simulink model "IEEE30_case"  (R2024b)
settings: Solver=FixedStepAuto  StartTime=0  StopTime=5  FixedStep=1e-7  RelTol=1e-3
values from neighbouring files (symbols this model uses):
  GFL_DFIG_7_C_bus = 0.08    [IEEE30_case_parameters.m]
  GFL_DFIG_7_D_mutual = 2.500000e+3    (= 2500)    [IEEE30_case_parameters.m]
  GFL_DFIG_7_f0 = 60    [IEEE30_case_parameters.m]
  GFL_DFIG_7_gPLLi = 3200    [IEEE30_case_parameters.m]
  GFL_DFIG_7_gPLLp = 650    [IEEE30_case_parameters.m]
  GFL_DFIG_7_H_WT = 0.4    [IEEE30_case_parameters.m]
  GFL_DFIG_7_Hg = 0.8    [IEEE30_case_parameters.m]
  GFL_DFIG_7_Igq_ref = 0    [IEEE30_case_parameters.m]
  GFL_DFIG_7_Ird_ref = 704.45696    [IEEE30_case_parameters.m]
  GFL_DFIG_7_KI_V = -300000    [IEEE30_case_parameters.m]
  GFL_DFIG_7_KP_V = -1000    [IEEE30_case_parameters.m]
  GFL_DFIG_7_Ksh = 1.254300e+4    (= 12543)    [IEEE30_case_parameters.m]
  GFL_DFIG_7_Lg = 0.000483    [IEEE30_case_parameters.m]
  GFL_DFIG_7_Lm_pu = 4    [IEEE30_case_parameters.m]
  GFL_DFIG_7_N = 100    [IEEE30_case_parameters.m]
  GFL_DFIG_7_p = 2    [IEEE30_case_parameters.m]
  GFL_DFIG_7_Pitch = 0    [IEEE30_case_parameters.m]
  GFL_DFIG_7_R = 44    [IEEE30_case_parameters.m]
  GFL_DFIG_7_Rg = 2.000000e-5    (= 2e-05)    [IEEE30_case_parameters.m]
  GFL_DFIG_7_rho = 1.225    [IEEE30_case_parameters.m]
  GFL_DFIG_7_rPLLi = 4500    [IEEE30_case_parameters.m]
  GFL_DFIG_7_rPLLp = 620    [IEEE30_case_parameters.m]
  GFL_DFIG_7_Rs_pu = 0.011    [IEEE30_case_parameters.m]
  GFL_DFIG_7_Sbase = 2.000000e+6    (= 2000000)    [IEEE30_case_parameters.m]
  GFL_DFIG_7_ugq_ref = 0    [IEEE30_case_parameters.m]
  GFL_DFIG_7_usd_ref = 0    [IEEE30_case_parameters.m]
  GFL_DFIG_7_Vbase = 690    [IEEE30_case_parameters.m]
  GFL_DFIG_7_Vdc_ref = 1200    [IEEE30_case_parameters.m]
  GFL_DFIG_7_wind = 12    [IEEE30_case_parameters.m]
  GFL_DFIG_7_wm_ref = 518.184209    [IEEE30_case_parameters.m]
  SG_D_13_D = 0.01056    [IEEE30_case_parameters.m]
  SG_D_13_EnableSaturation = 0    [IEEE30_case_parameters.m]
  SG_D_13_f0 = 60    [IEEE30_case_parameters.m]
  SG_D_13_H = 7.5    [IEEE30_case_parameters.m]
  SG_D_13_K_A = 20    [IEEE30_case_parameters.m]
  SG_D_13_K_E = 1.000000e+1    (= 10)    [IEEE30_case_parameters.m]
  SG_D_13_K_F = 2.363    [IEEE30_case_parameters.m]
  SG_D_13_K_s = 0.5    [IEEE30_case_parameters.m]
  SG_D_13_R_a = 0.001088    [IEEE30_case_parameters.m]
  SG_D_13_S_A = 1    [IEEE30_case_parameters.m]
  SG_D_13_S_B = 0.103    [IEEE30_case_parameters.m]
  SG_D_13_S_N = 10.659857    [IEEE30_case_parameters.m]
  SG_D_13_SpeedPara = 200    [IEEE30_case_parameters.m]
  SG_D_13_T_0 = 0.370163    [IEEE30_case_parameters.m]
  SG_D_13_T_1 = 0.3    [IEEE30_case_parameters.m]
  SG_D_13_T_2 = 0.05    [IEEE30_case_parameters.m]
  SG_D_13_T_3 = 0.02    [IEEE30_case_parameters.m]
  SG_D_13_T_4 = 0.005    [IEEE30_case_parameters.m]
  SG_D_13_T_A = 0.02    [IEEE30_case_parameters.m]
  SG_D_13_T_dd = 8.000000e+0    (= 8)    [IEEE30_case_parameters.m]
  SG_D_13_T_ddd = 0.04    [IEEE30_case_parameters.m]
  SG_D_13_T_E = 0.314    [IEEE30_case_parameters.m]
  SG_D_13_T_F = 0.35    [IEEE30_case_parameters.m]
  SG_D_13_T_qd = 0.8    [IEEE30_case_parameters.m]
  SG_D_13_T_qdd = 0.02    [IEEE30_case_parameters.m]
  SG_D_13_T_speed = 0.1    [IEEE30_case_parameters.m]
  SG_D_13_T_w = 0.5    [IEEE30_case_parameters.m]
  SG_D_13_V_ref = 1.696619    [IEEE30_case_parameters.m]
  SG_D_13_w_ref = 376.991118    [IEEE30_case_parameters.m]
  SG_D_13_x_d = 1.9    [IEEE30_case_parameters.m]
  SG_D_13_x_dd = 0.302    [IEEE30_case_parameters.m]
  SG_D_13_x_ddd = 0.204    [IEEE30_case_parameters.m]
  SG_D_13_x_l = 0.05    [IEEE30_case_parameters.m]
  SG_D_13_x_q = 1.3    [IEEE30_case_parameters.m]
  SG_D_13_x_qd = 0.5    [IEEE30_case_parameters.m]
  SG_D_13_x_qdd = 0.3    [IEEE30_case_parameters.m]
  SG_D_1_D = 0.01056    [IEEE30_case_parameters.m]
  SG_D_1_EnableSaturation = 0    [IEEE30_case_parameters.m]
  SG_D_1_f0 = 60    [IEEE30_case_parameters.m]
  SG_D_1_H = 7.5    [IEEE30_case_parameters.m]
  SG_D_1_K_A = 20    [IEEE30_case_parameters.m]
  SG_D_1_K_E = 1.000000e+1    (= 10)    [IEEE30_case_parameters.m]
  SG_D_1_K_F = 2.363    [IEEE30_case_parameters.m]
  SG_D_1_K_s = 0.5    [IEEE30_case_parameters.m]
  SG_D_1_R_a = 0.001088    [IEEE30_case_parameters.m]
  SG_D_1_S_A = 1    [IEEE30_case_parameters.m]
  SG_D_1_S_B = 0.103    [IEEE30_case_parameters.m]
  SG_D_1_S_N = 10.659857    [IEEE30_case_parameters.m]
  SG_D_1_SpeedPara = 200    [IEEE30_case_parameters.m]
  SG_D_1_T_0 = 0.259812    [IEEE30_case_parameters.m]
  SG_D_1_T_1 = 0.3    [IEEE30_case_parameters.m]
  SG_D_1_T_2 = 0.05    [IEEE30_case_parameters.m]
  SG_D_1_T_3 = 0.02    [IEEE30_case_parameters.m]
  SG_D_1_T_4 = 0.005    [IEEE30_case_parameters.m]
  SG_D_1_T_A = 0.02    [IEEE30_case_parameters.m]
  SG_D_1_T_dd = 8.000000e+0    (= 8)    [IEEE30_case_parameters.m]
  SG_D_1_T_ddd = 0.04    [IEEE30_case_parameters.m]
  SG_D_1_T_E = 0.314    [IEEE30_case_parameters.m]
  SG_D_1_T_F = 0.35    [IEEE30_case_parameters.m]
  SG_D_1_T_qd = 0.8    [IEEE30_case_parameters.m]
  SG_D_1_T_qdd = 0.02    [IEEE30_case_parameters.m]
  SG_D_1_T_speed = 0.1    [IEEE30_case_parameters.m]
  SG_D_1_T_w = 0.5    [IEEE30_case_parameters.m]
  SG_D_1_V_ref = 1.544107    [IEEE30_case_parameters.m]
  SG_D_1_w_ref = 376.991118    [IEEE30_case_parameters.m]
  SG_D_1_x_d = 1.9    [IEEE30_case_parameters.m]
  SG_D_1_x_dd = 0.302    [IEEE30_case_parameters.m]
  SG_D_1_x_ddd = 0.204    [IEEE30_case_parameters.m]
  SG_D_1_x_l = 0.05    [IEEE30_case_parameters.m]
  SG_D_1_x_q = 1.3    [IEEE30_case_parameters.m]
  SG_D_1_x_qd = 0.5    [IEEE30_case_parameters.m]
  SG_D_1_x_qdd = 0.3    [IEEE30_case_parameters.m]
  SG_D_22_D = 0.01056    [IEEE30_case_parameters.m]
  SG_D_22_EnableSaturation = 0    [IEEE30_case_parameters.m]
  SG_D_22_f0 = 60    [IEEE30_case_parameters.m]
  SG_D_22_H = 7.5    [IEEE30_case_parameters.m]
  SG_D_22_K_A = 20    [IEEE30_case_parameters.m]
  SG_D_22_K_E = 1.000000e+1    (= 10)    [IEEE30_case_parameters.m]
  SG_D_22_K_F = 2.363    [IEEE30_case_parameters.m]
  SG_D_22_K_s = 0.5    [IEEE30_case_parameters.m]
  SG_D_22_R_a = 0.001088    [IEEE30_case_parameters.m]
  SG_D_22_S_A = 1    [IEEE30_case_parameters.m]
  SG_D_22_S_B = 0.103    [IEEE30_case_parameters.m]
  SG_D_22_S_N = 10.659857    [IEEE30_case_parameters.m]
  SG_D_22_SpeedPara = 200    [IEEE30_case_parameters.m]
  SG_D_22_T_0 = 0.216121    [IEEE30_case_parameters.m]
  SG_D_22_T_1 = 0.3    [IEEE30_case_parameters.m]
  SG_D_22_T_2 = 0.05    [IEEE30_case_parameters.m]
  SG_D_22_T_3 = 0.02    [IEEE30_case_parameters.m]
  SG_D_22_T_4 = 0.005    [IEEE30_case_parameters.m]
  ... (+126 more)
(part 2 of 27)

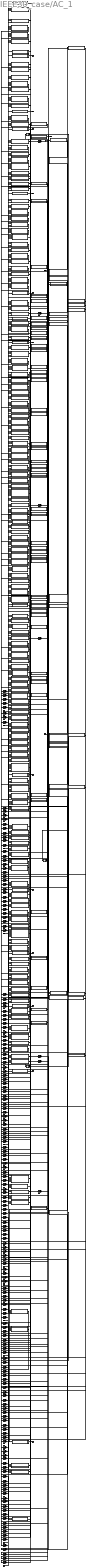
== system IEEE30_case/AC_1 ==
  id_SG_D_1 : Inport
  iq_SG_D_1 : Inport  Port=2
  id_SG_D_2 : Inport  Port=3
  iq_SG_D_2 : Inport  Port=4
  id_GFL_DFIG_7 : Inport  Port=5
  iq_GFL_DFIG_7 : Inport  Port=6
  id_SG_D_13 : Inport  Port=7
  iq_SG_D_13 : Inport  Port=8
  id_SG_D_22 : Inport  Port=9
  iq_SG_D_22 : Inport  Port=10
  id_SG_D_23 : Inport  Port=11
  iq_SG_D_23 : Inport  Port=12
  id_SG_D_27 : Inport  Port=13
  iq_SG_D_27 : Inport  Port=14
  d_id_line_10_17_block : Subsystem
  d_id_line_10_20_block : Subsystem
  d_id_line_10_21_block : Subsystem
  d_id_line_10_22_block : Subsystem
  d_id_line_12_13_block : Subsystem
  d_id_line_12_14_block : Subsystem
  d_id_line_12_15_block : Subsystem
  d_id_line_12_16_block : Subsystem
  d_id_line_14_15_block : Subsystem
  d_id_line_15_18_block : Subsystem
  d_id_line_15_23_block : Subsystem
  d_id_line_16_17_block : Subsystem
  d_id_line_18_19_block : Subsystem
  d_id_line_19_20_block : Subsystem
  d_id_line_1_2_block : Subsystem
  d_id_line_1_3_block : Subsystem
  d_id_line_21_22_block : Subsystem
  d_id_line_22_24_block : Subsystem
  d_id_line_23_24_block : Subsystem
  d_id_line_24_25_block : Subsystem
  d_id_line_25_26_block : Subsystem
  d_id_line_25_27_block : Subsystem
  d_id_line_27_29_block : Subsystem
  d_id_line_27_30_block : Subsystem
  d_id_line_28_27_block : Subsystem
  d_id_line_29_30_block : Subsystem
  d_id_line_2_4_block : Subsystem
  d_id_line_2_5_block : Subsystem
  d_id_line_2_6_block : Subsystem
  d_id_line_3_4_block : Subsystem
  d_id_line_4_12_block : Subsystem
  d_id_line_4_6_block : Subsystem
  d_id_line_5_7_block : Subsystem
  d_id_line_6_10_block : Subsystem
  d_id_line_6_28_block : Subsystem
  d_id_line_6_7_block : Subsystem
  d_id_line_6_8_block : Subsystem
  d_id_line_6_9_block : Subsystem
  d_id_line_8_28_block : Subsystem
  d_id_line_9_10_block : Subsystem
  d_id_line_9_11_block : Subsystem
  d_id_load_10_block : Subsystem
  d_id_load_12_block : Subsystem
  d_id_load_14_block : Subsystem
  d_id_load_15_block : Subsystem
  d_id_load_16_block : Subsystem
  d_id_load_17_block : Subsystem
  d_id_load_18_block : Subsystem
  d_id_load_19_block : Subsystem
  d_id_load_20_block : Subsystem
  d_id_load_21_block : Subsystem
  d_id_load_23_block : Subsystem
  d_id_load_24_block : Subsystem
  d_id_load_26_block : Subsystem
  d_id_load_29_block : Subsystem
  d_id_load_2_block : Subsystem
  d_id_load_30_block : Subsystem
  d_id_load_3_block : Subsystem
  d_id_load_4_block : Subsystem
  d_id_load_7_block : Subsystem
  d_id_load_8_block : Subsystem
  d_iq_line_10_17_block : Subsystem
  d_iq_line_10_20_block : Subsystem
  d_iq_line_10_21_block : Subsystem
  d_iq_line_10_22_block : Subsystem
  d_iq_line_12_13_block : Subsystem
  d_iq_line_12_14_block : Subsystem
  d_iq_line_12_15_block : Subsystem
  d_iq_line_12_16_block : Subsystem
  d_iq_line_14_15_block : Subsystem
  d_iq_line_15_18_block : Subsystem
  d_iq_line_15_23_block : Subsystem
  d_iq_line_16_17_block : Subsystem
  d_iq_line_18_19_block : Subsystem
  d_iq_line_19_20_block : Subsystem
  d_iq_line_1_2_block : Subsystem
  d_iq_line_1_3_block : Subsystem
  d_iq_line_21_22_block : Subsystem
  d_iq_line_22_24_block : Subsystem
  d_iq_line_23_24_block : Subsystem
  d_iq_line_24_25_block : Subsystem
  d_iq_line_25_26_block : Subsystem
  d_iq_line_25_27_block : Subsystem
  d_iq_line_27_29_block : Subsystem
  d_iq_line_27_30_block : Subsystem
  d_iq_line_28_27_block : Subsystem
  d_iq_line_29_30_block : Subsystem
  d_iq_line_2_4_block : Subsystem
  d_iq_line_2_5_block : Subsystem
  d_iq_line_2_6_block : Subsystem
  d_iq_line_3_4_block : Subsystem
  d_iq_line_4_12_block : Subsystem
  d_iq_line_4_6_block : Subsystem
  d_iq_line_5_7_block : Subsystem
  d_iq_line_6_10_block : Subsystem
  d_iq_line_6_28_block : Subsystem
  d_iq_line_6_7_block : Subsystem
  d_iq_line_6_8_block : Subsystem
  d_iq_line_6_9_block : Subsystem
  d_iq_line_8_28_block : Subsystem
  d_iq_line_9_10_block : Subsystem
  d_iq_line_9_11_block : Subsystem
  d_iq_load_10_block : Subsystem
  d_iq_load_12_block : Subsystem
  d_iq_load_14_block : Subsystem
  d_iq_load_15_block : Subsystem
  d_iq_load_16_block : Subsystem
  d_iq_load_17_block : Subsystem
  d_iq_load_18_block : Subsystem
  d_iq_load_19_block : Subsystem
  d_iq_load_20_block : Subsystem
  d_iq_load_21_block : Subsystem
  d_iq_load_23_block : Subsystem
  d_iq_load_24_block : Subsystem
  d_iq_load_26_block : Subsystem
  d_iq_load_29_block : Subsystem
  d_iq_load_2_block : Subsystem
  d_iq_load_30_block : Subsystem
  d_iq_load_3_block : Subsystem
  d_iq_load_4_block : Subsystem
  d_iq_load_7_block : Subsystem
  d_iq_load_8_block : Subsystem
  d_vd_bus_10_block : Subsystem
  d_vd_bus_11_block : Subsystem
  d_vd_bus_12_block : Subsystem
  d_vd_bus_13_block : Subsystem
  d_vd_bus_14_block : Subsystem
  d_vd_bus_15_block : Subsystem
  d_vd_bus_16_block : Subsystem
  d_vd_bus_17_block : Subsystem
  d_vd_bus_18_block : Subsystem
  d_vd_bus_19_block : Subsystem
  d_vd_bus_1_block : Subsystem
  d_vd_bus_20_block : Subsystem
  d_vd_bus_21_block : Subsystem
  d_vd_bus_22_block : Subsystem
  d_vd_bus_23_block : Subsystem
  d_vd_bus_24_block : Subsystem
  d_vd_bus_25_block : Subsystem
  d_vd_bus_26_block : Subsystem
  d_vd_bus_27_block : Subsystem
  d_vd_bus_28_block : Subsystem
  d_vd_bus_29_block : Subsystem
  d_vd_bus_2_block : Subsystem
  d_vd_bus_30_block : Subsystem
  d_vd_bus_3_block : Subsystem
  d_vd_bus_4_block : Subsystem
  d_vd_bus_5_block : Subsystem
  d_vd_bus_6_block : Subsystem
  d_vd_bus_7_block : Subsystem
  d_vd_bus_8_block : Subsystem
  d_vd_bus_9_block : Subsystem
  d_vq_bus_10_block : Subsystem
  d_vq_bus_11_block : Subsystem
  d_vq_bus_12_block : Subsystem
  d_vq_bus_13_block : Subsystem
  d_vq_bus_14_block : Subsystem
  d_vq_bus_15_block : Subsystem
  d_vq_bus_16_block : Subsystem
  d_vq_bus_17_block : Subsystem
  d_vq_bus_18_block : Subsystem
  d_vq_bus_19_block : Subsystem
  d_vq_bus_1_block : Subsystem
  d_vq_bus_20_block : Subsystem
  d_vq_bus_21_block : Subsystem
  d_vq_bus_22_block : Subsystem
  d_vq_bus_23_block : Subsystem
  d_vq_bus_24_block : Subsystem
  d_vq_bus_25_block : Subsystem
  d_vq_bus_26_block : Subsystem
  d_vq_bus_27_block : Subsystem
  d_vq_bus_28_block : Subsystem
  d_vq_bus_29_block : Subsystem
  d_vq_bus_2_block : Subsystem
  d_vq_bus_30_block : Subsystem
  d_vq_bus_3_block : Subsystem
  d_vq_bus_4_block : Subsystem
  d_vq_bus_5_block : Subsystem
  d_vq_bus_6_block : Subsystem
  d_vq_bus_7_block : Subsystem
  d_vq_bus_8_block : Subsystem
  d_vq_bus_9_block : Subsystem
  id_bus_10_block : Subsystem
  id_bus_11_block : Subsystem
  id_bus_12_block : Subsystem
  id_bus_13_block : Subsystem
  id_bus_14_block : Subsystem
  id_bus_15_block : Subsystem
  id_bus_16_block : Subsystem
  id_bus_17_block : Subsystem
  id_bus_18_block : Subsystem
  id_bus_19_block : Subsystem
  id_bus_1_block : Subsystem
  id_bus_20_block : Subsystem
  id_bus_21_block : Subsystem
  id_bus_22_block : Subsystem
  id_bus_23_block : Subsystem
  id_bus_24_block : Subsystem
  id_bus_25_block : Subsystem
  id_bus_26_block : Subsystem
  id_bus_27_block : Subsystem
  id_bus_28_block : Subsystem
  id_bus_29_block : Subsystem
  id_bus_2_block : Subsystem
  id_bus_30_block : Subsystem
  id_bus_3_block : Subsystem
  id_bus_4_block : Subsystem
  id_bus_5_block : Subsystem
  id_bus_6_block : Subsystem
  id_bus_7_block : Subsystem
  id_bus_8_block : Subsystem
  id_bus_9_block : Subsystem
  id_line_10_17 : Integrator  InitialCondition=0.0294
  id_line_10_20 : Integrator  InitialCondition=0.0572
  id_line_10_21 : Integrator  InitialCondition=-0.0157
  id_line_10_22 : Integrator  InitialCondition=-0.033
  id_line_12_13 : Integrator  InitialCondition=-0.3728
  id_line_12_14 : Integrator  InitialCondition=0.0544
  id_line_12_15 : Integrator  InitialCondition=0.0964
  id_line_12_16 : Integrator  InitialCondition=0.094
  id_line_14_15 : Integrator  InitialCondition=-0.0084
  id_line_15_18 : Integrator  InitialCondition=0.0931
  id_line_15_23 : Integrator  InitialCondition=-0.0876
  id_line_16_17 : Integrator  InitialCondition=0.0591
  id_line_18_19 : Integrator  InitialCondition=0.0607
  id_line_19_20 : Integrator  InitialCondition=-0.0351
  id_line_1_2 : Integrator  InitialCondition=0.1089
  id_line_1_3 : Integrator  InitialCondition=0.1508
  id_line_21_22 : Integrator  InitialCondition=-0.1847
  id_line_22_24 : Integrator  InitialCondition=-0.0256
  id_line_23_24 : Integrator  InitialCondition=0.0706
  id_line_24_25 : Integrator  InitialCondition=-0.0398
  id_line_25_26 : Integrator  InitialCondition=0.0351
  id_line_25_27 : Integrator  InitialCondition=-0.0749
  id_line_27_29 : Integrator  InitialCondition=0.0615
  id_line_27_30 : Integrator  InitialCondition=0.071
  id_line_28_27 : Integrator  InitialCondition=-0.0602
  id_line_29_30 : Integrator  InitialCondition=0.0373
  id_line_2_4 : Integrator  InitialCondition=0.1602
  id_line_2_5 : Integrator  InitialCondition=0.1375
  id_line_2_6 : Integrator  InitialCondition=0.2021
  id_line_3_4 : Integrator  InitialCondition=0.1265
  id_line_4_12 : Integrator  InitialCondition=-0.0164
  id_line_4_6 : Integrator  InitialCondition=0.2258
  id_line_5_7 : Integrator  InitialCondition=0.137
  id_line_6_10 : Integrator  InitialCondition=0.0347
  id_line_6_28 : Integrator  InitialCondition=-0.007
  id_line_6_7 : Integrator  InitialCondition=0.0937
  id_line_6_8 : Integrator  InitialCondition=0.2449
  id_line_6_9 : Integrator  InitialCondition=0.0608
  id_line_8_28 : Integrator  InitialCondition=-0.0526
  id_line_9_10 : Integrator  InitialCondition=0.0608
  id_line_9_11 : Integrator  InitialCondition=0.0
  id_load_10 : Integrator  InitialCondition=0.05762064982199419
  id_load_12 : Integrator  InitialCondition=0.11156942833231305
  id_load_14 : Integrator  InitialCondition=0.06276933195309545
  id_load_15 : Integrator  InitialCondition=0.08255703677859036
  id_load_16 : Integrator  InitialCondition=0.03492161173939187
  id_load_17 : Integrator  InitialCondition=0.08845667800489554
  id_load_18 : Integrator  InitialCondition=0.03241810454985263
  id_load_19 : Integrator  InitialCondition=0.09575018801243466
  id_load_2 : Integrator  InitialCondition=0.21607333892385353
  id_load_20 : Integrator  InitialCondition=0.02216052273204651
  id_load_21 : Integrator  InitialCondition=0.16897904373299158
  id_load_23 : Integrator  InitialCondition=0.031543951844660426
  id_load_24 : Integrator  InitialCondition=0.08480178555101445
  id_load_26 : Integrator  InitialCondition=0.03509280097479722
  id_load_29 : Integrator  InitialCondition=0.024141745519164363
  id_load_3 : Integrator  InitialCondition=0.024078796739266696
  id_load_30 : Integrator  InitialCondition=0.10832152401242767
  id_load_4 : Integrator  InitialCondition=0.07699434378766279
  id_load_7 : Integrator  InitialCondition=0.33349238327258734
  id_load_8 : Integrator  InitialCondition=0.29709225448369286
  iq_bus_10_block : Subsystem
  iq_bus_11_block : Subsystem
  iq_bus_12_block : Subsystem
  iq_bus_13_block : Subsystem
  iq_bus_14_block : Subsystem
  iq_bus_15_block : Subsystem
  iq_bus_16_block : Subsystem
  iq_bus_17_block : Subsystem
  iq_bus_18_block : Subsystem
  iq_bus_19_block : Subsystem
  iq_bus_1_block : Subsystem
  iq_bus_20_block : Subsystem
  iq_bus_21_block : Subsystem
  iq_bus_22_block : Subsystem
  iq_bus_23_block : Subsystem
  iq_bus_24_block : Subsystem
  iq_bus_25_block : Subsystem
  iq_bus_26_block : Subsystem
  iq_bus_27_block : Subsystem
  iq_bus_28_block : Subsystem
  iq_bus_29_block : Subsystem
  iq_bus_2_block : Subsystem
  iq_bus_30_block : Subsystem
  iq_bus_3_block : Subsystem
  iq_bus_4_block : Subsystem
  iq_bus_5_block : Subsystem
  iq_bus_6_block : Subsystem
  iq_bus_7_block : Subsystem
  iq_bus_8_block : Subsystem
  iq_bus_9_block : Subsystem
  iq_line_10_17 : Integrator  InitialCondition=-0.0833
  iq_line_10_20 : Integrator  InitialCondition=-0.0504
  iq_line_10_21 : Integrator  InitialCondition=0.1196
  iq_line_10_22 : Integrator  InitialCondition=0.0883
  iq_line_12_13 : Integrator  InitialCondition=0.104
  iq_line_12_14 : Integrator  InitialCondition=-0.0104
  iq_line_12_15 : Integrator  InitialCondition=0.0082
  iq_line_12_16 : Integrator  InitialCondition=-0.0015
  iq_line_14_15 : Integrator  InitialCondition=0.0085
  iq_line_15_18 : Integrator  InitialCondition=-0.0115
  iq_line_15_23 : Integrator  InitialCondition=0.0571
  iq_line_16_17 : Integrator  InitialCondition=0.0186
  iq_line_18_19 : Integrator  InitialCondition=-0.0002
  iq_line_19_20 : Integrator  InitialCondition=0.0417
  iq_line_1_2 : Integrator  InitialCondition=0.0359
  iq_line_1_3 : Integrator  InitialCondition=-0.0509
  iq_line_21_22 : Integrator  InitialCondition=0.2429
  iq_line_22_24 : Integrator  InitialCondition=-0.0766
  iq_line_23_24 : Integrator  InitialCondition=-0.0108
  iq_line_24_25 : Integrator  InitialCondition=-0.0161
  iq_line_25_26 : Integrator  InitialCondition=-0.025
  iq_line_25_27 : Integrator  InitialCondition=0.0089
  iq_line_27_29 : Integrator  InitialCondition=-0.0177
  iq_line_27_30 : Integrator  InitialCondition=-0.0178
  iq_line_28_27 : Integrator  InitialCondition=0.0649
  iq_line_29_30 : Integrator  InitialCondition=-0.0076
  iq_line_2_4 : Integrator  InitialCondition=-0.0632
  iq_line_2_5 : Integrator  InitialCondition=-0.0561
  iq_line_2_6 : Integrator  InitialCondition=-0.0857
  iq_line_3_4 : Integrator  InitialCondition=-0.0479
  iq_line_4_12 : Integrator  InitialCondition=0.0212
  iq_line_4_6 : Integrator  InitialCondition=-0.1233
  iq_line_5_7 : Integrator  InitialCondition=-0.0727
  iq_line_6_10 : Integrator  InitialCondition=0.0183
  iq_line_6_28 : Integrator  InitialCondition=0.0232
  iq_line_6_7 : Integrator  InitialCondition=-0.0411
  iq_line_6_8 : Integrator  InitialCondition=-0.2609
  iq_line_6_9 : Integrator  InitialCondition=0.0321
  iq_line_8_28 : Integrator  InitialCondition=0.0563
  iq_line_9_10 : Integrator  InitialCondition=0.0321
  iq_line_9_11 : Integrator  InitialCondition=0.0
  iq_load_10 : Integrator  InitialCondition=-0.023750155710290172
  iq_load_12 : Integrator  InitialCondition=-0.07912681099168954
  iq_load_14 : Integrator  InitialCondition=-0.018925276841010825
  iq_load_15 : Integrator  InitialCondition=-0.028857933169465035
  iq_load_16 : Integrator  InitialCondition=-0.02004887361778872
  iq_load_17 : Integrator  InitialCondition=-0.06472122976436909
  iq_load_18 : Integrator  InitialCondition=-0.011280947855116687
  iq_load_19 : Integrator  InitialCondition=-0.041932223185470595
  iq_load_2 : Integrator  InitialCondition=-0.12857026174935463
  iq_load_20 : Integrator  InitialCondition=-0.008738712343444175
  iq_load_21 : Integrator  InitialCondition=-0.12325613888050702
  iq_load_23 : Integrator  InitialCondition=-0.016881324060089138
  iq_load_24 : Integrator  InitialCondition=-0.07174395043107668
  iq_load_26 : Integrator  InitialCondition=-0.024985253536549745
  iq_load_29 : Integrator  InitialCondition=-0.010091059482716875
  iq_load_3 : Integrator  InitialCondition=-0.01284992759642887
  iq_load_30 : Integrator  InitialCondition=-0.025413778164099808
  iq_load_4 : Integrator  InitialCondition=-0.018745546356930477
  iq_load_7 : Integrator  InitialCondition=-0.1282452809846534
  iq_load_8 : Integrator  InitialCondition=-0.3267952741267314
  vd_bus_1 : Integrator  InitialCondition=1.0
  vd_bus_10 : Integrator  InitialCondition=0.9826970239916736
  vd_bus_11 : Integrator  InitialCondition=0.9791651158395024
  vd_bus_12 : Integrator  InitialCondition=0.9851138013134092
  vd_bus_13 : Integrator  InitialCondition=0.9996681288543109
  vd_bus_13_out_block : Subsystem
  vd_bus_14 : Integrator  InitialCondition=0.9758845077744954
  vd_bus_15 : Integrator  InitialCondition=0.9794312058156106
  vd_bus_16 : Integrator  InitialCondition=0.9763547800086462
  vd_bus_17 : Integrator  InitialCondition=0.9751536962265143
  vd_bus_18 : Integrator  InitialCondition=0.9666562258898125
  vd_bus_19 : Integrator  InitialCondition=0.9629845116632844
  vd_bus_1_out_block : Subsystem
  vd_bus_2 : Integrator  InitialCondition=0.9999737066760137
  vd_bus_20 : Integrator  InitialCondition=0.96695524349606
  vd_bus_21 : Integrator  InitialCondition=0.9915427046125346
  vd_bus_22 : Integrator  InitialCondition=0.998247346015286
  vd_bus_22_out_block : Subsystem
  vd_bus_23 : Integrator  InitialCondition=0.9996153468676248
  vd_bus_23_out_block : Subsystem
  vd_bus_24 : Integrator  InitialCondition=0.9875238668019122
  vd_bus_25 : Integrator  InitialCondition=0.9897841246173575
  vd_bus_26 : Integrator  InitialCondition=0.9715165251247116
  vd_bus_27 : Integrator  InitialCondition=0.9998954705679283
  vd_bus_27_out_block : Subsystem
  vd_bus_28 : Integrator  InitialCondition=0.9739527539680385
  vd_bus_29 : Integrator  InitialCondition=0.9789208214366218
  vd_bus_2_out_block : Subsystem
  vd_bus_3 : Integrator  InitialCondition=0.9827914051679246
  vd_bus_30 : Integrator  InitialCondition=0.9665194654171512
  vd_bus_4 : Integrator  InitialCondition=0.9796122119954275
  vd_bus_5 : Integrator  InitialCondition=0.9818864593128205
  vd_bus_6 : Integrator  InitialCondition=0.9724223804183465
  vd_bus_7 : Integrator  InitialCondition=0.9663195284431091
  vd_bus_7_out_block : Subsystem
  vd_bus_8 : Integrator  InitialCondition=0.9595368480969235
  vd_bus_9 : Integrator  InitialCondition=0.9791651158395024
  vq_bus_1 : Integrator  InitialCondition=0.0
  vq_bus_10 : Integrator  InitialCondition=-0.05795157371804589
  vq_bus_11 : Integrator  InitialCondition=-0.051263313202214764
  vq_bus_12 : Integrator  InitialCondition=-0.026431197200791515
  vq_bus_13 : Integrator  InitialCondition=0.02576105884704402
  vq_bus_13_out_block : Subsystem
  vq_bus_14 : Integrator  InitialCondition=-0.039332654939370465
  vq_bus_15 : Integrator  InitialCondition=-0.03954066677889769
  vq_bus_16 : Integrator  InitialCondition=-0.04509567319714669
  vq_bus_17 : Integrator  InitialCondition=-0.057803961717475
  vq_bus_18 : Integrator  InitialCondition=-0.05875724397019161
  vq_bus_19 : Integrator  InitialCondition=-0.0666325737803011
  vq_bus_1_out_block : Subsystem
  vq_bus_2 : Integrator  InitialCondition=-0.007251617518437124
  vq_bus_20 : Integrator  InitialCondition=-0.06542912996363182
  vq_bus_21 : Integrator  InitialCondition=-0.06044373953148359
  vq_bus_22 : Integrator  InitialCondition=-0.059179693928221304
  vq_bus_22_out_block : Subsystem
  vq_bus_23 : Integrator  InitialCondition=-0.02773370344397317
  vq_bus_23_out_block : Subsystem
  vq_bus_24 : Integrator  InitialCondition=-0.045386583835857836
  vq_bus_25 : Integrator  InitialCondition=-0.029203013743050087
  vq_bus_26 : Integrator  InitialCondition=-0.036291964728132654
  vq_bus_27 : Integrator  InitialCondition=-0.014458490161195933
  vq_bus_27_out_block : Subsystem
  vq_bus_28 : Integrator  InitialCondition=-0.03853789459848076
  vq_bus_29 : Integrator  InitialCondition=-0.036382963166013
  vq_bus_2_out_block : Subsystem
  vq_bus_3 : Integrator  InitialCondition=-0.026114195223675894
  vq_bus_30 : Integrator  InitialCondition=-0.05135554854968241
  vq_bus_4 : Integrator  InitialCondition=-0.030695321441965278
  vq_bus_5 : Integrator  InitialCondition=-0.03195188283298677
  vq_bus_6 : Integrator  InitialCondition=-0.038494815818198067
  vq_bus_7 : Integrator  InitialCondition=-0.04475640282897933
  vq_bus_7_out_block : Subsystem
  vq_bus_8 : Integrator  InitialCondition=-0.04568314085508728
  vq_bus_9 : Integrator  InitialCondition=-0.051263313202214764
  vd_bus_1_out : Outport
  vq_bus_1_out : Outport  Port=2
  vd_bus_2_out : Outport  Port=3
  vq_bus_2_out : Outport  Port=4
  vd_bus_7_out : Outport  Port=5
  vq_bus_7_out : Outport  Port=6
  vd_bus_13_out : Outport  Port=7
  vq_bus_13_out : Outport  Port=8
  vd_bus_22_out : Outport  Port=9
  vq_bus_22_out : Outport  Port=10
  vd_bus_23_out : Outport  Port=11
  vq_bus_23_out : Outport  Port=12
  vd_bus_27_out : Outport  Port=13
  vq_bus_27_out : Outport  Port=14
  wires:
  id_line_2_6/1 -> id_bus_6_block/1(State_id_line_2_6_f1c81), id_bus_2_block/6(State_id_line_2_6_b437f), d_id_line_2_6_block/1(State_id_line_2_6_7d8f0), d_iq_line_2_6_block/1(State_id_line_2_6_7b42f)
  id_SG_D_27/1 -> id_bus_27_block/1(Input_id_SG_D_27_bfa21)
  iq_line_27_29/1 -> d_id_line_27_29_block/2(State_iq_line_27_29_70df7), d_iq_line_27_29_block/2(State_iq_line_27_29_e2b12), iq_bus_27_block/3(State_iq_line_27_29_e7090), iq_bus_29_block/2(State_iq_line_27_29_eb40a)
  iq_line_2_5/1 -> d_id_line_2_5_block/2(State_iq_line_2_5_6b567), iq_bus_2_block/5(State_iq_line_2_5_9d19f), d_iq_line_2_5_block/2(State_iq_line_2_5_e8b89), iq_bus_5_block/1(State_iq_line_2_5_98d2b)
  iq_SG_D_27/1 -> iq_bus_27_block/1(Input_iq_SG_D_27_5f248)
  id_bus_4_block/1(Blockout_id_bus_4_62c4e) -> d_vd_bus_4_block/1(Alge_id_bus_4_472b5)
  id_line_12_13/1 -> d_iq_line_12_13_block/1(State_id_line_12_13_e0b57), id_bus_12_block/3(State_id_line_12_13_02bcf), id_bus_13_block/2(State_id_line_12_13_e1ea8)
  iq_line_28_27/1 -> iq_bus_27_block/5(State_iq_line_28_27_c8698), iq_bus_28_block/3(State_iq_line_28_27_5cab2), d_id_line_28_27_block/1(State_iq_line_28_27_dccca)
  id_load_19/1 -> d_iq_load_19_block/1(State_id_load_19_a4f80), d_id_load_19_block/1(State_id_load_19_86caa), id_bus_19_block/1(State_id_load_19_6dd0b)
  iq_load_19/1 -> d_id_load_19_block/2(State_iq_load_19_76cc3), iq_bus_19_block/1(State_iq_load_19_c9423), d_iq_load_19_block/2(State_iq_load_19_a3943)
  d_id_line_22_24_block/1(Blockout_d_id_line_22_24_ad4cf) -> id_line_22_24/1
  iq_line_1_2/1 -> iq_bus_1_block/2(State_iq_line_1_2_426df), iq_bus_2_block/3(State_iq_line_1_2_22297), d_id_line_1_2_block/2(State_iq_line_1_2_034b5), d_iq_line_1_2_block/2(State_iq_line_1_2_62f2c)
  iq_GFL_DFIG_7/1 -> iq_bus_7_block/1(Input_iq_GFL_DFIG_7_603eb)
  id_bus_10_block/1(Blockout_id_bus_10_f7cfc) -> d_vd_bus_10_block/1(Alge_id_bus_10_55824)
  vq_bus_25/1 -> d_iq_line_25_26_block/3(State_vq_bus_25_a69b5), d_iq_line_24_25_block/4(State_vq_bus_25_584b4), d_vd_bus_25_block/2(State_vq_bus_25_926f5), d_iq_line_25_27_block/3(State_vq_bus_25_cd5c7)
  d_vq_bus_26_block/1(Blockout_d_vq_bus_26_2e68a) -> vq_bus_26/1
  iq_SG_D_23/1 -> iq_bus_23_block/1(Input_iq_SG_D_23_15e34)
  iq_SG_D_22/1 -> iq_bus_22_block/1(Input_iq_SG_D_22_7afaf)
  iq_bus_13_block/1(Blockout_iq_bus_13_72f64) -> d_vq_bus_13_block/1(Alge_iq_bus_13_8e98b)
  id_bus_9_block/1(Blockout_id_bus_9_0b36c) -> d_vd_bus_9_block/1(Alge_id_bus_9_9bb77)
  d_id_load_4_block/1(Blockout_d_id_load_4_41d2b) -> id_load_4/1
  id_bus_12_block/1(Blockout_id_bus_12_a7f7d) -> d_vd_bus_12_block/1(Alge_id_bus_12_e0ed8)
  d_vd_bus_21_block/1(Blockout_d_vd_bus_21_3eacf) -> vd_bus_21/1
  d_iq_line_6_28_block/1(Blockout_d_iq_line_6_28_5907d) -> iq_line_6_28/1
  id_line_27_30/1 -> d_id_line_27_30_block/1(State_id_line_27_30_d82b5), d_iq_line_27_30_block/1(State_id_line_27_30_d18cd), id_bus_30_block/2(State_id_line_27_30_55115), id_bus_27_block/4(State_id_line_27_30_1b75b)
  id_bus_25_block/1(Blockout_id_bus_25_a9e73) -> d_vd_bus_25_block/1(Alge_id_bus_25_c584c)
  vd_bus_2_out_block/1(Blockout_vd_bus_2_out_6e542) -> vd_bus_2_out/1
  d_id_load_16_block/1(Blockout_d_id_load_16_4c50d) -> id_load_16/1
  iq_load_4/1 -> d_id_load_4_block/2(State_iq_load_4_59598), iq_bus_4_block/1(State_iq_load_4_0a7a4), d_iq_load_4_block/2(State_iq_load_4_cbd44)
  d_vq_bus_13_block/1(Blockout_d_vq_bus_13_29628) -> vq_bus_13/1
  id_load_18/1 -> id_bus_18_block/1(State_id_load_18_b6089), d_id_load_18_block/1(State_id_load_18_c255f), d_iq_load_18_block/1(State_id_load_18_cc435)
  iq_line_25_27/1 -> iq_bus_27_block/2(State_iq_line_25_27_786f4), iq_bus_25_block/3(State_iq_line_25_27_6cee1), d_id_line_25_27_block/2(State_iq_line_25_27_73a3b), d_iq_line_25_27_block/2(State_iq_line_25_27_e5d71)
  id_bus_18_block/1(Blockout_id_bus_18_f6aba) -> d_vd_bus_18_block/1(Alge_id_bus_18_7cead)
  d_iq_load_7_block/1(Blockout_d_iq_load_7_f7ad2) -> iq_load_7/1
  d_vd_bus_18_block/1(Blockout_d_vd_bus_18_c0af9) -> vd_bus_18/1
  d_iq_line_4_12_block/1(Blockout_d_iq_line_4_12_9b276) -> iq_line_4_12/1
  id_line_1_2/1 -> d_iq_line_1_2_block/1(State_id_line_1_2_bca8d), id_bus_1_block/2(State_id_line_1_2_dfc68), d_id_line_1_2_block/1(State_id_line_1_2_ffdd4), id_bus_2_block/3(State_id_line_1_2_35b9f)
  id_line_1_3/1 -> d_id_line_1_3_block/1(State_id_line_1_3_6eb6f), id_bus_1_block/3(State_id_line_1_3_6e2c0), id_bus_3_block/2(State_id_line_1_3_85a3c), d_iq_line_1_3_block/1(State_id_line_1_3_ae183)
  id_GFL_DFIG_7/1 -> id_bus_7_block/1(Input_id_GFL_DFIG_7_848f8)
  id_SG_D_13/1 -> id_bus_13_block/1(Input_id_SG_D_13_a3cac)
  d_id_line_6_8_block/1(Blockout_d_id_line_6_8_230ec) -> id_line_6_8/1
  iq_bus_19_block/1(Blockout_iq_bus_19_07988) -> d_vq_bus_19_block/1(Alge_iq_bus_19_ec54b)
  iq_bus_21_block/1(Blockout_iq_bus_21_51471) -> d_vq_bus_21_block/1(Alge_iq_bus_21_81fa7)
  d_iq_load_8_block/1(Blockout_d_iq_load_8_09960) -> iq_load_8/1
  id_bus_6_block/1(Blockout_id_bus_6_41f21) -> d_vd_bus_6_block/1(Alge_id_bus_6_cc19e)
  iq_load_26/1 -> d_iq_load_26_block/2(State_iq_load_26_73904), iq_bus_26_block/1(State_iq_load_26_ac2a5), d_id_load_26_block/2(State_iq_load_26_8de5f)
  id_SG_D_22/1 -> id_bus_22_block/1(Input_id_SG_D_22_c72e9)
  d_vq_bus_14_block/1(Blockout_d_vq_bus_14_01909) -> vq_bus_14/1
  id_bus_3_block/1(Blockout_id_bus_3_36e80) -> d_vd_bus_3_block/1(Alge_id_bus_3_320e9)
  id_SG_D_23/1 -> id_bus_23_block/1(Input_id_SG_D_23_b9b6b)
  d_iq_line_19_20_block/1(Blockout_d_iq_line_19_20_abe71) -> iq_line_19_20/1
  d_id_line_9_10_block/1(Blockout_d_id_line_9_10_c8100) -> id_line_9_10/1
  vq_bus_28/1 -> d_vd_bus_28_block/2(State_vq_bus_28_2c3ac), d_iq_line_28_27_block/3(State_vq_bus_28_55731), d_iq_line_6_28_block/3(State_vq_bus_28_c063c), d_iq_line_8_28_block/3(State_vq_bus_28_2fdab)
  vq_bus_29/1 -> d_vd_bus_29_block/2(State_vq_bus_29_f75e0), d_iq_line_29_30_block/3(State_vq_bus_29_3e7b3), d_iq_load_29_block/3(State_vq_bus_29_603a8), d_iq_line_27_29_block/4(State_vq_bus_29_394c9)
  vq_bus_16/1 -> d_vd_bus_16_block/2(State_vq_bus_16_133e3), d_iq_line_12_16_block/4(State_vq_bus_16_185e6), d_iq_load_16_block/3(State_vq_bus_16_c51f8), d_iq_line_16_17_block/3(State_vq_bus_16_312ae)
  iq_bus_8_block/1(Blockout_iq_bus_8_3c8c0) -> d_vq_bus_8_block/1(Alge_iq_bus_8_bb8a6)
  d_id_line_16_17_block/1(Blockout_d_id_line_16_17_1cf66) -> id_line_16_17/1
  iq_line_2_6/1 -> d_id_line_2_6_block/2(State_iq_line_2_6_13ccb), iq_bus_2_block/6(State_iq_line_2_6_42b8c), iq_bus_6_block/1(State_iq_line_2_6_0b501), d_iq_line_2_6_block/2(State_iq_line_2_6_17b05)
  iq_line_6_28/1 -> iq_bus_6_block/7(State_iq_line_6_28_c6c23), d_iq_line_6_28_block/2(State_iq_line_6_28_bd7e8), d_id_line_6_28_block/2(State_iq_line_6_28_4e6de), iq_bus_28_block/1(State_iq_line_6_28_9fc56)
  id_SG_D_1/1 -> id_bus_1_block/1(Input_id_SG_D_1_df3b6)
  id_load_29/1 -> d_id_load_29_block/1(State_id_load_29_75998), id_bus_29_block/1(State_id_load_29_01b75), d_iq_load_29_block/1(State_id_load_29_0ee5a)
  id_line_22_24/1 -> d_id_line_22_24_block/1(State_id_line_22_24_bf52a), id_bus_24_block/2(State_id_line_22_24_03003), d_iq_line_22_24_block/1(State_id_line_22_24_f3c92), id_bus_22_block/4(State_id_line_22_24_1a6a9)
  d_id_line_18_19_block/1(Blockout_d_id_line_18_19_39807) -> id_line_18_19/1
  iq_load_14/1 -> d_id_load_14_block/2(State_iq_load_14_d649f), d_iq_load_14_block/2(State_iq_load_14_32f4c), iq_bus_14_block/1(State_iq_load_14_72e79)
  iq_bus_28_block/1(Blockout_iq_bus_28_fc1de) -> d_vq_bus_28_block/1(Alge_iq_bus_28_e3380)
  vd_bus_1/1 -> d_vq_bus_1_block/2(State_vd_bus_1_0a414), vd_bus_1_out_block/1(State_vd_bus_1_2d719), d_id_line_1_2_block/3(State_vd_bus_1_c4c37), d_id_line_1_3_block/3(State_vd_bus_1_5ec44)
  d_iq_load_18_block/1(Blockout_d_iq_load_18_ea1d4) -> iq_load_18/1
  d_vq_bus_3_block/1(Blockout_d_vq_bus_3_10f19) -> vq_bus_3/1
  d_iq_line_22_24_block/1(Blockout_d_iq_line_22_24_c0f91) -> iq_line_22_24/1
  iq_SG_D_13/1 -> iq_bus_13_block/1(Input_iq_SG_D_13_41b6f)
  d_id_line_10_21_block/1(Blockout_d_id_line_10_21_8be6c) -> id_line_10_21/1
  vq_bus_2/1 -> d_vd_bus_2_block/2(State_vq_bus_2_2b9b5), d_iq_line_1_2_block/4(State_vq_bus_2_54dcd), d_iq_line_2_5_block/3(State_vq_bus_2_03b90), vq_bus_2_out_block/1(State_vq_bus_2_331ca), d_iq_line_2_4_block/3(State_vq_bus_2_08b2a), d_iq_line_2_6_block/3(State_vq_bus_2_0704f), d_iq_load_2_block/3(State_vq_bus_2_2efc8)
  vd_bus_29/1 -> d_vq_bus_29_block/2(State_vd_bus_29_8221e), d_id_line_29_30_block/3(State_vd_bus_29_072b3), d_id_line_27_29_block/4(State_vd_bus_29_a9de4), d_id_load_29_block/3(State_vd_bus_29_01a46)
  d_vd_bus_16_block/1(Blockout_d_vd_bus_16_30db1) -> vd_bus_16/1
  iq_bus_30_block/1(Blockout_iq_bus_30_f5578) -> d_vq_bus_30_block/1(Alge_iq_bus_30_b84d2)
  iq_line_8_28/1 -> d_id_line_8_28_block/2(State_iq_line_8_28_05745), d_iq_line_8_28_block/2(State_iq_line_8_28_65df2), iq_bus_8_block/3(State_iq_line_8_28_57c78), iq_bus_28_block/2(State_iq_line_8_28_5df2a)
  id_load_24/1 -> d_id_load_24_block/1(State_id_load_24_1ae10), d_iq_load_24_block/1(State_id_load_24_9d769), id_bus_24_block/1(State_id_load_24_1483c)
  id_load_14/1 -> d_id_load_14_block/1(State_id_load_14_cc3a3), d_iq_load_14_block/1(State_id_load_14_258e7), id_bus_14_block/1(State_id_load_14_8acb6)
  d_iq_load_30_block/1(Blockout_d_iq_load_30_29807) -> iq_load_30/1
  iq_line_22_24/1 -> d_id_line_22_24_block/2(State_iq_line_22_24_ef354), iq_bus_22_block/4(State_iq_line_22_24_573df), iq_bus_24_block/2(State_iq_line_22_24_76281), d_iq_line_22_24_block/2(State_iq_line_22_24_cd212)
  d_iq_load_26_block/1(Blockout_d_iq_load_26_2c5ef) -> iq_load_26/1
  vq_bus_27/1 -> d_vd_bus_27_block/2(State_vq_bus_27_1ff45), d_iq_line_25_27_block/4(State_vq_bus_27_3c154), d_iq_line_27_29_block/3(State_vq_bus_27_cc3b8), d_iq_line_27_30_block/3(State_vq_bus_27_cb66b), vq_bus_27_out_block/1(State_vq_bus_27_50cd3), d_iq_line_28_27_block/2(State_vq_bus_27_b0dc4)
  id_bus_16_block/1(Blockout_id_bus_16_3e58c) -> d_vd_bus_16_block/1(Alge_id_bus_16_f0bf0)
  id_line_14_15/1 -> d_id_line_14_15_block/1(State_id_line_14_15_28cb1), d_iq_line_14_15_block/1(State_id_line_14_15_7494d), id_bus_15_block/3(State_id_line_14_15_22f97), id_bus_14_block/3(State_id_line_14_15_8760d)
  d_id_line_10_20_block/1(Blockout_d_id_line_10_20_f93f3) -> id_line_10_20/1
  iq_bus_29_block/1(Blockout_iq_bus_29_54fcd) -> d_vq_bus_29_block/1(Alge_iq_bus_29_a773e)
  vq_bus_20/1 -> d_iq_line_19_20_block/4(State_vq_bus_20_72c0e), d_vd_bus_20_block/2(State_vq_bus_20_f55e8), d_iq_load_20_block/3(State_vq_bus_20_5757f), d_iq_line_10_20_block/4(State_vq_bus_20_32cb1)
  d_iq_line_9_11_block/1(Blockout_d_iq_line_9_11_ec45f) -> iq_line_9_11/1
  d_iq_line_25_26_block/1(Blockout_d_iq_line_25_26_d7e2d) -> iq_line_25_26/1
  d_vq_bus_10_block/1(Blockout_d_vq_bus_10_d65a2) -> vq_bus_10/1
  id_bus_20_block/1(Blockout_id_bus_20_0c62a) -> d_vd_bus_20_block/1(Alge_id_bus_20_5519e)
  iq_load_30/1 -> iq_bus_30_block/1(State_iq_load_30_e4c4c), d_id_load_30_block/2(State_iq_load_30_241a5), d_iq_load_30_block/2(State_iq_load_30_a149a)
  iq_SG_D_1/1 -> iq_bus_1_block/1(Input_iq_SG_D_1_636be)
  iq_SG_D_2/1 -> iq_bus_2_block/1(Input_iq_SG_D_2_3deae)
  id_line_10_22/1 -> id_bus_10_block/7(State_id_line_10_22_301e1), id_bus_22_block/2(State_id_line_10_22_83f91), d_id_line_10_22_block/1(State_id_line_10_22_89fbc), d_iq_line_10_22_block/1(State_id_line_10_22_084f6)
  id_SG_D_2/1 -> id_bus_2_block/1(Input_id_SG_D_2_271b9)
  id_load_8/1 -> d_id_load_8_block/1(State_id_load_8_d111e), d_iq_load_8_block/1(State_id_load_8_a69c1), id_bus_8_block/1(State_id_load_8_2d300)
  iq_line_10_22/1 -> d_id_line_10_22_block/2(State_iq_line_10_22_73dd3), iq_bus_10_block/7(State_iq_line_10_22_b2379), d_iq_line_10_22_block/2(State_iq_line_10_22_3080a), iq_bus_22_block/2(State_iq_line_10_22_172f8)
  id_bus_19_block/1(Blockout_id_bus_19_c959d) -> d_vd_bus_19_block/1(Alge_id_bus_19_2b5fc)
  id_load_15/1 -> d_id_load_15_block/1(State_id_load_15_eb719), id_bus_15_block/1(State_id_load_15_060ab), d_iq_load_15_block/1(State_id_load_15_529a5)
  iq_line_23_24/1 -> d_id_line_23_24_block/2(State_iq_line_23_24_865cb), iq_bus_23_block/4(State_iq_line_23_24_17ece), iq_bus_24_block/3(State_iq_line_23_24_946d1), d_iq_line_23_24_block/2(State_iq_line_23_24_146a4)
  id_load_2/1 -> d_id_load_2_block/1(State_id_load_2_b9eb3), d_iq_load_2_block/1(State_id_load_2_4fe58), id_bus_2_block/2(State_id_load_2_17a4a)
  iq_line_19_20/1 -> d_id_line_19_20_block/2(State_iq_line_19_20_aecba), iq_bus_19_block/3(State_iq_line_19_20_3626a), d_iq_line_19_20_block/2(State_iq_line_19_20_2451d), iq_bus_20_block/3(State_iq_line_19_20_435ec)
  id_bus_30_block/1(Blockout_id_bus_30_50341) -> d_vd_bus_30_block/1(Alge_id_bus_30_9d0e0)
  id_bus_7_block/1(Blockout_id_bus_7_1a1e5) -> d_vd_bus_7_block/1(Alge_id_bus_7_b77de)
  id_bus_11_block/1(Blockout_id_bus_11_04e0f) -> d_vd_bus_11_block/1(Alge_id_bus_11_02d21)
  vd_bus_30/1 -> d_id_load_30_block/3(State_vd_bus_30_c111a), d_id_line_29_30_block/4(State_vd_bus_30_f5954), d_id_line_27_30_block/4(State_vd_bus_30_fc433), d_vq_bus_30_block/2(State_vd_bus_30_536bd)
  iq_bus_14_block/1(Blockout_iq_bus_14_40877) -> d_vq_bus_14_block/1(Alge_iq_bus_14_fa60c)
  iq_line_18_19/1 -> d_iq_line_18_19_block/2(State_iq_line_18_19_da0b4), iq_bus_18_block/3(State_iq_line_18_19_1de76), iq_bus_19_block/2(State_iq_line_18_19_b0a61), d_id_line_18_19_block/2(State_iq_line_18_19_bad0a)
  id_line_5_7/1 -> d_id_line_5_7_block/1(State_id_line_5_7_f4de4), d_iq_line_5_7_block/1(State_id_line_5_7_c3a9a), id_bus_5_block/2(State_id_line_5_7_98a48), id_bus_7_block/3(State_id_line_5_7_86c29)
  id_bus_22_block/1(Blockout_id_bus_22_34fe4) -> d_vd_bus_22_block/1(Alge_id_bus_22_6e14d)
  iq_load_7/1 -> d_iq_load_7_block/2(State_iq_load_7_42ee7), iq_bus_7_block/2(State_iq_load_7_52d26), d_id_load_7_block/2(State_iq_load_7_25d21)
  id_bus_15_block/1(Blockout_id_bus_15_03e1f) -> d_vd_bus_15_block/1(Alge_id_bus_15_5fc28)
  id_bus_29_block/1(Blockout_id_bus_29_dcea9) -> d_vd_bus_29_block/1(Alge_id_bus_29_eb4d1)
  d_vd_bus_28_block/1(Blockout_d_vd_bus_28_2c5eb) -> vd_bus_28/1
  iq_line_1_3/1 -> iq_bus_1_block/3(State_iq_line_1_3_a1a02), iq_bus_3_block/2(State_iq_line_1_3_704f9), d_iq_line_1_3_block/2(State_iq_line_1_3_f4510), d_id_line_1_3_block/2(State_iq_line_1_3_e0dcf)
  d_iq_load_16_block/1(Blockout_d_iq_load_16_0762f) -> iq_load_16/1
  iq_load_15/1 -> d_iq_load_15_block/2(State_iq_load_15_0f08a), iq_bus_15_block/1(State_iq_load_15_d1891), d_id_load_15_block/2(State_iq_load_15_a3946)
  iq_line_6_7/1 -> d_iq_line_6_7_block/2(State_iq_line_6_7_562f8), iq_bus_7_block/4(State_iq_line_6_7_6dde0), d_id_line_6_7_block/2(State_iq_line_6_7_8098b), iq_bus_6_block/3(State_iq_line_6_7_5270c)
  id_bus_28_block/1(Blockout_id_bus_28_5bbbe) -> d_vd_bus_28_block/1(Alge_id_bus_28_5e372)
  d_iq_load_24_block/1(Blockout_d_iq_load_24_ad216) -> iq_load_24/1
  d_vq_bus_22_block/1(Blockout_d_vq_bus_22_04fe2) -> vq_bus_22/1
  d_iq_line_12_15_block/1(Blockout_d_iq_line_12_15_872fa) -> iq_line_12_15/1
  id_line_15_23/1 -> d_iq_line_15_23_block/1(State_id_line_15_23_e0160), d_id_line_15_23_block/1(State_id_line_15_23_5b9f7), id_bus_15_block/5(State_id_line_15_23_df0bc), id_bus_23_block/3(State_id_line_15_23_e01a5)
  iq_bus_27_block/1(Blockout_iq_bus_27_6c5f3) -> d_vq_bus_27_block/1(Alge_iq_bus_27_548e5)
  iq_load_29/1 -> d_iq_load_29_block/2(State_iq_load_29_c7734), iq_bus_29_block/1(State_iq_load_29_82b4e), d_id_load_29_block/2(State_iq_load_29_726f9)
  id_bus_27_block/1(Blockout_id_bus_27_09b01) -> d_vd_bus_27_block/1(Alge_id_bus_27_de3da)
  vd_bus_7/1 -> d_vq_bus_7_block/2(State_vd_bus_7_0bd1f), d_id_load_7_block/3(State_vd_bus_7_efc9a), vd_bus_7_out_block/1(State_vd_bus_7_01f81), d_id_line_5_7_block/4(State_vd_bus_7_ca274), d_id_line_6_7_block/4(State_vd_bus_7_fcdb6)
  vd_bus_26/1 -> d_id_load_26_block/3(State_vd_bus_26_1ef7d), d_id_line_25_26_block/4(State_vd_bus_26_fc271), d_vq_bus_26_block/2(State_vd_bus_26_21468)
  iq_line_12_16/1 -> d_iq_line_12_16_block/2(State_iq_line_12_16_057ef), iq_bus_16_block/2(State_iq_line_12_16_8d22f), iq_bus_12_block/6(State_iq_line_12_16_bc787), d_id_line_12_16_block/2(State_iq_line_12_16_288fb)
  vd_bus_13_out_block/1(Blockout_vd_bus_13_out_de49d) -> vd_bus_13_out/1
  iq_bus_17_block/1(Blockout_iq_bus_17_f1a33) -> d_vq_bus_17_block/1(Alge_iq_bus_17_e57db)
  iq_bus_26_block/1(Blockout_iq_bus_26_d1a08) -> d_vq_bus_26_block/1(Alge_iq_bus_26_172b0)
  d_iq_line_6_8_block/1(Blockout_d_iq_line_6_8_b8ba9) -> iq_line_6_8/1
  vd_bus_6/1 -> d_vq_bus_6_block/2(State_vd_bus_6_1a151), d_id_line_4_6_block/4(State_vd_bus_6_4e65f), d_id_line_6_10_block/3(State_vd_bus_6_f8a31), d_id_line_6_7_block/3(State_vd_bus_6_7185e), d_id_line_2_6_block/4(State_vd_bus_6_4e456), d_id_line_6_8_block/3(State_vd_bus_6_a2a00), d_id_line_6_28_block/4(State_vd_bus_6_24f43), d_id_line_6_9_block/2(State_vd_bus_6_dd441)
  vd_bus_4/1 -> d_vq_bus_4_block/2(State_vd_bus_4_783ad), d_id_line_2_4_block/4(State_vd_bus_4_468ae), d_id_line_4_6_block/3(State_vd_bus_4_4594e), d_id_line_4_12_block/3(State_vd_bus_4_83c34), d_id_load_4_block/3(State_vd_bus_4_a96c2), d_id_line_3_4_block/4(State_vd_bus_4_76476)
  iq_bus_20_block/1(Blockout_iq_bus_20_faa95) -> d_vq_bus_20_block/1(Alge_iq_bus_20_dac44)
  d_vd_bus_30_block/1(Blockout_d_vd_bus_30_d4924) -> vd_bus_30/1
  vq_bus_4/1 -> d_vd_bus_4_block/2(State_vq_bus_4_40a27), d_iq_line_4_6_block/3(State_vq_bus_4_bd5e4), d_iq_load_4_block/3(State_vq_bus_4_cd35f), d_iq_line_2_4_block/4(State_vq_bus_4_bf96b), d_iq_line_4_12_block/3(State_vq_bus_4_bbada), d_iq_line_3_4_block/4(State_vq_bus_4_f5988)
  id_bus_1_block/1(Blockout_id_bus_1_c8a02) -> d_vd_bus_1_block/1(Alge_id_bus_1_1678c)
  id_bus_21_block/1(Blockout_id_bus_21_f6b53) -> d_vd_bus_21_block/1(Alge_id_bus_21_08784)
  d_vq_bus_28_block/1(Blockout_d_vq_bus_28_fc78f) -> vq_bus_28/1
  vq_bus_14/1 -> d_iq_load_14_block/3(State_vq_bus_14_0c5a3), d_iq_line_14_15_block/3(State_vq_bus_14_61922), d_vd_bus_14_block/2(State_vq_bus_14_a6726), d_iq_line_12_14_block/4(State_vq_bus_14_44cc5)
  id_bus_26_block/1(Blockout_id_bus_26_f258d) -> d_vd_bus_26_block/1(Alge_id_bus_26_ff4d0)
  iq_bus_25_block/1(Blockout_iq_bus_25_a2b76) -> d_vq_bus_25_block/1(Alge_iq_bus_25_b52f0)
  id_bus_13_block/1(Blockout_id_bus_13_e8139) -> d_vd_bus_13_block/1(Alge_id_bus_13_da285)
  iq_bus_24_block/1(Blockout_iq_bus_24_a8f54) -> d_vq_bus_24_block/1(Alge_iq_bus_24_0b825)
  iq_bus_4_block/1(Blockout_iq_bus_4_c8ef1) -> d_vq_bus_4_block/1(Alge_iq_bus_4_edea5)
  id_bus_24_block/1(Blockout_id_bus_24_85e6b) -> d_vd_bus_24_block/1(Alge_id_bus_24_d1ab9)
  d_iq_line_12_14_block/1(Blockout_d_iq_line_12_14_a9efb) -> iq_line_12_14/1
  vq_bus_23_out_block/1(Blockout_vq_bus_23_out_e2230) -> vq_bus_23_out/1
  iq_bus_23_block/1(Blockout_iq_bus_23_896ad) -> d_vq_bus_23_block/1(Alge_iq_bus_23_4fd9f)
  d_id_line_28_27_block/1(Blockout_d_id_line_28_27_ed70c) -> id_line_28_27/1
  id_bus_17_block/1(Blockout_id_bus_17_5f54e) -> d_vd_bus_17_block/1(Alge_id_bus_17_92d80)
  iq_line_9_10/1 -> d_id_line_9_10_block/1(State_iq_line_9_10_60482), iq_bus_10_block/3(State_iq_line_9_10_547ec), iq_bus_9_block/2(State_iq_line_9_10_59358)
  id_bus_23_block/1(Blockout_id_bus_23_84113) -> d_vd_bus_23_block/1(Alge_id_bus_23_3d01a)
  iq_line_15_23/1 -> d_id_line_15_23_block/2(State_iq_line_15_23_b33ff), iq_bus_15_block/5(State_iq_line_15_23_dd72a), iq_bus_23_block/3(State_iq_line_15_23_fc0a9), d_iq_line_15_23_block/2(State_iq_line_15_23_ade94)
  iq_bus_22_block/1(Blockout_iq_bus_22_6516e) -> d_vq_bus_22_block/1(Alge_iq_bus_22_4e114)
  d_id_line_23_24_block/1(Blockout_d_id_line_23_24_092ff) -> id_line_23_24/1
  vd_bus_17/1 -> d_vq_bus_17_block/2(State_vd_bus_17_b3717), d_id_line_16_17_block/4(State_vd_bus_17_81d16), d_id_line_10_17_block/4(State_vd_bus_17_0c9ca), d_id_load_17_block/3(State_vd_bus_17_34bc4)
  iq_line_24_25/1 -> d_id_line_24_25_block/2(State_iq_line_24_25_5d4c8), d_iq_line_24_25_block/2(State_iq_line_24_25_774ec), iq_bus_24_block/4(State_iq_line_24_25_99c0f), iq_bus_25_block/1(State_iq_line_24_25_0047e)
  iq_bus_18_block/1(Blockout_iq_bus_18_b4916) -> d_vq_bus_18_block/1(Alge_iq_bus_18_aa760)
  id_load_3/1 -> d_iq_load_3_block/1(State_id_load_3_67436), id_bus_3_block/1(State_id_load_3_6a44d), d_id_load_3_block/1(State_id_load_3_6ca3f)
  vd_bus_3/1 -> d_vq_bus_3_block/2(State_vd_bus_3_2475d), d_id_line_1_3_block/4(State_vd_bus_3_137a9), d_id_load_3_block/3(State_vd_bus_3_703c2), d_id_line_3_4_block/3(State_vd_bus_3_9cd0a)
  id_load_10/1 -> d_iq_load_10_block/1(State_id_load_10_13915), id_bus_10_block/1(State_id_load_10_705f8), d_id_load_10_block/1(State_id_load_10_b4421)
  id_line_6_10/1 -> d_iq_line_6_10_block/1(State_id_line_6_10_fd3de), id_bus_10_block/2(State_id_line_6_10_65dc9), id_bus_6_block/6(State_id_line_6_10_2c687)
  iq_bus_16_block/1(Blockout_iq_bus_16_0845b) -> d_vq_bus_16_block/1(Alge_iq_bus_16_974ba)
  d_vd_bus_8_block/1(Blockout_d_vd_bus_8_6724c) -> vd_bus_8/1
  iq_line_9_11/1 -> iq_bus_9_block/3(State_iq_line_9_11_56031), iq_bus_11_block/1(State_iq_line_9_11_5dafe), d_id_line_9_11_block/1(State_iq_line_9_11_d1a32)
  id_line_28_27/1 -> id_bus_27_block/5(State_id_line_28_27_22b40), id_bus_28_block/3(State_id_line_28_27_48f21), d_iq_line_28_27_block/1(State_id_line_28_27_3a5d8)
  iq_bus_12_block/1(Blockout_iq_bus_12_94dfd) -> d_vq_bus_12_block/1(Alge_iq_bus_12_c8c41)
  vq_bus_6/1 -> d_vd_bus_6_block/2(State_vq_bus_6_b1fab), d_iq_line_6_9_block/2(State_vq_bus_6_65d52), d_iq_line_6_10_block/3(State_vq_bus_6_fa482), d_iq_line_2_6_block/4(State_vq_bus_6_e98dc), d_iq_line_6_7_block/3(State_vq_bus_6_83d07), d_iq_line_4_6_block/4(State_vq_bus_6_b2fe0), d_iq_line_6_28_block/4(State_vq_bus_6_177ff), d_iq_line_6_8_block/3(State_vq_bus_6_241ca)
  d_vd_bus_6_block/1(Blockout_d_vd_bus_6_cb8a2) -> vd_bus_6/1
  iq_bus_15_block/1(Blockout_iq_bus_15_ccbd2) -> d_vq_bus_15_block/1(Alge_iq_bus_15_10184)
  d_iq_load_10_block/1(Blockout_d_iq_load_10_a5f74) -> iq_load_10/1
  id_line_10_21/1 -> id_bus_10_block/6(State_id_line_10_21_c8fce), id_bus_21_block/2(State_id_line_10_21_bcd00), d_iq_line_10_21_block/1(State_id_line_10_21_eaa10), d_id_line_10_21_block/1(State_id_line_10_21_d3f7b)
  d_id_line_9_11_block/1(Blockout_d_id_line_9_11_6700a) -> id_line_9_11/1
  vd_bus_9/1 -> d_id_line_9_11_block/3(State_vd_bus_9_653b8), d_id_line_9_10_block/3(State_vd_bus_9_a12d0), d_id_line_6_9_block/3(State_vd_bus_9_1e8eb), d_vq_bus_9_block/2(State_vd_bus_9_08774)
  id_bus_14_block/1(Blockout_id_bus_14_a7723) -> d_vd_bus_14_block/1(Alge_id_bus_14_c396c)
  d_vq_bus_6_block/1(Blockout_d_vq_bus_6_ac6cf) -> vq_bus_6/1
  d_iq_load_12_block/1(Blockout_d_iq_load_12_fd87b) -> iq_load_12/1
  d_vd_bus_9_block/1(Blockout_d_vd_bus_9_ffce9) -> vd_bus_9/1
  vd_bus_22_out_block/1(Blockout_vd_bus_22_out_b1115) -> vd_bus_22_out/1
  iq_bus_11_block/1(Blockout_iq_bus_11_40b0f) -> d_vq_bus_11_block/1(Alge_iq_bus_11_6efd4)
  id_line_6_9/1 -> id_bus_9_block/1(State_id_line_6_9_06348), id_bus_6_block/5(State_id_line_6_9_c95db), d_iq_line_6_9_block/1(State_id_line_6_9_7cf57)
  id_bus_2_block/1(Blockout_id_bus_2_bbec8) -> d_vd_bus_2_block/1(Alge_id_bus_2_79afc)
  id_load_26/1 -> d_id_load_26_block/1(State_id_load_26_7d329), id_bus_26_block/1(State_id_load_26_80bb7), d_iq_load_26_block/1(State_id_load_26_7e9e7)
  d_vq_bus_5_block/1(Blockout_d_vq_bus_5_f1f0c) -> vq_bus_5/1
  d_iq_line_2_6_block/1(Blockout_d_iq_line_2_6_890b3) -> iq_line_2_6/1
  iq_bus_10_block/1(Blockout_iq_bus_10_f080b) -> d_vq_bus_10_block/1(Alge_iq_bus_10_74e9d)
  d_vq_bus_12_block/1(Blockout_d_vq_bus_12_c4166) -> vq_bus_12/1
  iq_line_15_18/1 -> iq_bus_15_block/4(State_iq_line_15_18_a2738), d_id_line_15_18_block/2(State_iq_line_15_18_872e9), d_iq_line_15_18_block/2(State_iq_line_15_18_85966), iq_bus_18_block/2(State_iq_line_15_18_3f1e8)
  d_iq_line_23_24_block/1(Blockout_d_iq_line_23_24_07ba5) -> iq_line_23_24/1
  vd_bus_27_out_block/1(Blockout_vd_bus_27_out_73c03) -> vd_bus_27_out/1
  vd_bus_28/1 -> d_vq_bus_28_block/2(State_vd_bus_28_5e73c), d_id_line_28_27_block/3(State_vd_bus_28_9edc3), d_id_line_8_28_block/3(State_vd_bus_28_83ac0), d_id_line_6_28_block/3(State_vd_bus_28_34661)
  d_iq_line_25_27_block/1(Blockout_d_iq_line_25_27_06e15) -> iq_line_25_27/1
  id_bus_8_block/1(Blockout_id_bus_8_ac02c) -> d_vd_bus_8_block/1(Alge_id_bus_8_ddcea)
  vq_bus_10/1 -> d_iq_line_6_10_block/2(State_vq_bus_10_9c824), d_iq_line_10_20_block/3(State_vq_bus_10_01ccf), d_iq_load_10_block/3(State_vq_bus_10_c6f4b), d_iq_line_10_22_block/3(State_vq_bus_10_6b45e), d_vd_bus_10_block/2(State_vq_bus_10_0727d), d_iq_line_10_21_block/3(State_vq_bus_10_d2e20), d_iq_line_10_17_block/3(State_vq_bus_10_bd672), d_iq_line_9_10_block/2(State_vq_bus_10_72139)
  iq_bus_7_block/1(Blockout_iq_bus_7_06239) -> d_vq_bus_7_block/1(Alge_iq_bus_7_86528)
  iq_bus_6_block/1(Blockout_iq_bus_6_4f954) -> d_vq_bus_6_block/1(Alge_iq_bus_6_8f458)
  iq_bus_5_block/1(Blockout_iq_bus_5_aa6f8) -> d_vq_bus_5_block/1(Alge_iq_bus_5_20adf)
  id_bus_5_block/1(Blockout_id_bus_5_f0a59) -> d_vd_bus_5_block/1(Alge_id_bus_5_015f0)
  vq_bus_17/1 -> d_vd_bus_17_block/2(State_vq_bus_17_c3ce6), d_iq_line_10_17_block/4(State_vq_bus_17_4f180), d_iq_line_16_17_block/4(State_vq_bus_17_5c6e8), d_iq_load_17_block/3(State_vq_bus_17_aeaf0)
  d_id_line_10_17_block/1(Blockout_d_id_line_10_17_512b4) -> id_line_10_17/1
  d_id_line_10_22_block/1(Blockout_d_id_line_10_22_d0b41) -> id_line_10_22/1
  iq_load_24/1 -> d_id_load_24_block/2(State_iq_load_24_33ce7), d_iq_load_24_block/2(State_iq_load_24_562ce), iq_bus_24_block/1(State_iq_load_24_fdcb6)
  iq_bus_3_block/1(Blockout_iq_bus_3_0811d) -> d_vq_bus_3_block/1(Alge_iq_bus_3_cb5cd)
  iq_bus_2_block/1(Blockout_iq_bus_2_bb89e) -> d_vq_bus_2_block/1(Alge_iq_bus_2_6cf64)
  id_line_6_8/1 -> id_bus_6_block/4(State_id_line_6_8_8d48d), d_id_line_6_8_block/1(State_id_line_6_8_be2c2), d_iq_line_6_8_block/1(State_id_line_6_8_d622b), id_bus_8_block/2(State_id_line_6_8_e60f9)
  iq_bus_1_block/1(Blockout_iq_bus_1_c22d8) -> d_vq_bus_1_block/1(Alge_iq_bus_1_d0ef3)
  vd_bus_11/1 -> d_vq_bus_11_block/2(State_vd_bus_11_8616a), d_id_line_9_11_block/2(State_vd_bus_11_30158)
  iq_line_3_4/1 -> d_iq_line_3_4_block/2(State_iq_line_3_4_a2132), iq_bus_4_block/3(State_iq_line_3_4_5b109), iq_bus_3_block/3(State_iq_line_3_4_e67cb), d_id_line_3_4_block/2(State_iq_line_3_4_97dfa)
  id_line_25_26/1 -> d_iq_line_25_26_block/1(State_id_line_25_26_499e6), id_bus_26_block/2(State_id_line_25_26_45789), id_bus_25_block/2(State_id_line_25_26_94c65), d_id_line_25_26_block/1(State_id_line_25_26_99f78)
  vq_bus_27_out_block/1(Blockout_vq_bus_27_out_7c7b9) -> vq_bus_27_out/1
  id_line_15_18/1 -> d_id_line_15_18_block/1(State_id_line_15_18_9ff35), d_iq_line_15_18_block/1(State_id_line_15_18_c7b72), id_bus_18_block/2(State_id_line_15_18_185de), id_bus_15_block/4(State_id_line_15_18_9837d)
  vd_bus_23_out_block/1(Blockout_vd_bus_23_out_e84a6) -> vd_bus_23_out/1
  vd_bus_23/1 -> d_vq_bus_23_block/2(State_vd_bus_23_43c98), d_id_load_23_block/3(State_vd_bus_23_3d25c), d_id_line_23_24_block/3(State_vd_bus_23_dd709), d_id_line_15_23_block/4(State_vd_bus_23_ce9b8), vd_bus_23_out_block/1(State_vd_bus_23_a2fc7)
  iq_line_12_13/1 -> d_id_line_12_13_block/1(State_iq_line_12_13_e9023), iq_bus_13_block/2(State_iq_line_12_13_2e588), iq_bus_12_block/3(State_iq_line_12_13_64934)
  vq_bus_22_out_block/1(Blockout_vq_bus_22_out_dafa4) -> vq_bus_22_out/1
  vq_bus_13_out_block/1(Blockout_vq_bus_13_out_2bf25) -> vq_bus_13_out/1
  vd_bus_12/1 -> d_id_load_12_block/3(State_vd_bus_12_e073f), d_id_line_12_16_block/3(State_vd_bus_12_31adb), d_vq_bus_12_block/2(State_vd_bus_12_a627c), d_id_line_12_15_block/3(State_vd_bus_12_a4ba8), d_id_line_12_13_block/2(State_vd_bus_12_4b72e), d_id_line_4_12_block/2(State_vd_bus_12_eb3f5), d_id_line_12_14_block/3(State_vd_bus_12_691f6)
  iq_line_10_20/1 -> iq_bus_10_block/5(State_iq_line_10_20_d3f34), iq_bus_20_block/2(State_iq_line_10_20_d570b), d_iq_line_10_20_block/2(State_iq_line_10_20_af332), d_id_line_10_20_block/2(State_iq_line_10_20_a2259)
  id_line_21_22/1 -> d_iq_line_21_22_block/1(State_id_line_21_22_6fd19), id_bus_22_block/3(State_id_line_21_22_cc6ca), id_bus_21_block/3(State_id_line_21_22_cc9c2), d_id_line_21_22_block/1(State_id_line_21_22_e74c3)
  vq_bus_7_out_block/1(Blockout_vq_bus_7_out_1686e) -> vq_bus_7_out/1
  d_vd_bus_12_block/1(Blockout_d_vd_bus_12_8eaf3) -> vd_bus_12/1
  d_id_load_2_block/1(Blockout_d_id_load_2_a0af3) -> id_load_2/1
  vq_bus_23/1 -> d_vd_bus_23_block/2(State_vq_bus_23_506e6), vq_bus_23_out_block/1(State_vq_bus_23_75786), d_iq_load_23_block/3(State_vq_bus_23_fbc77), d_iq_line_23_24_block/3(State_vq_bus_23_d5a58), d_iq_line_15_23_block/4(State_vq_bus_23_32b73)
  vq_bus_1/1 -> d_vd_bus_1_block/2(State_vq_bus_1_acb41), d_iq_line_1_3_block/3(State_vq_bus_1_564cd), vq_bus_1_out_block/1(State_vq_bus_1_5ae62), d_iq_line_1_2_block/3(State_vq_bus_1_1d692)
  vq_bus_18/1 -> d_vd_bus_18_block/2(State_vq_bus_18_b1f41), d_iq_load_18_block/3(State_vq_bus_18_1cdbe), d_iq_line_15_18_block/4(State_vq_bus_18_6e5b1), d_iq_line_18_19_block/3(State_vq_bus_18_f4e53)
  vd_bus_7_out_block/1(Blockout_vd_bus_7_out_4e91c) -> vd_bus_7_out/1
  vq_bus_2_out_block/1(Blockout_vq_bus_2_out_9085b) -> vq_bus_2_out/1
  iq_line_27_30/1 -> d_id_line_27_30_block/2(State_iq_line_27_30_37807), d_iq_line_27_30_block/2(State_iq_line_27_30_e9a72), iq_bus_27_block/4(State_iq_line_27_30_e8aeb), iq_bus_30_block/2(State_iq_line_27_30_c3531)
  vq_bus_1_out_block/1(Blockout_vq_bus_1_out_7cf09) -> vq_bus_1_out/1
  iq_line_12_14/1 -> d_id_line_12_14_block/2(State_iq_line_12_14_78bfe), iq_bus_12_block/4(State_iq_line_12_14_05407), iq_bus_14_block/2(State_iq_line_12_14_c9961), d_iq_line_12_14_block/2(State_iq_line_12_14_89ecd)
  d_id_line_12_15_block/1(Blockout_d_id_line_12_15_9a1c2) -> id_line_12_15/1
  d_id_line_12_13_block/1(Blockout_d_id_line_12_13_70d92) -> id_line_12_13/1
  d_vq_bus_1_block/1(Blockout_d_vq_bus_1_b6261) -> vq_bus_1/1
  id_line_18_19/1 -> d_iq_line_18_19_block/1(State_id_line_18_19_8f9c3), id_bus_19_block/2(State_id_line_18_19_4e3a3), d_id_line_18_19_block/1(State_id_line_18_19_ee31e), id_bus_18_block/3(State_id_line_18_19_1fd25)
  d_vq_bus_7_block/1(Blockout_d_vq_bus_7_71b97) -> vq_bus_7/1
  vd_bus_1_out_block/1(Blockout_vd_bus_1_out_a0239) -> vd_bus_1_out/1
  iq_line_14_15/1 -> d_iq_line_14_15_block/2(State_iq_line_14_15_6bca3), d_id_line_14_15_block/2(State_iq_line_14_15_9579a), iq_bus_14_block/3(State_iq_line_14_15_62994), iq_bus_15_block/3(State_iq_line_14_15_cd3f2)
  vd_bus_27/1 -> d_vq_bus_27_block/2(State_vd_bus_27_e355a), d_id_line_25_27_block/4(State_vd_bus_27_199bb), d_id_line_27_30_block/3(State_vd_bus_27_614b7), d_id_line_27_29_block/3(State_vd_bus_27_91239), d_id_line_28_27_block/2(State_vd_bus_27_3c49b), vd_bus_27_out_block/1(State_vd_bus_27_9c8fe)
  iq_line_12_15/1 -> d_id_line_12_15_block/2(State_iq_line_12_15_08071), d_iq_line_12_15_block/2(State_iq_line_12_15_4b1af), iq_bus_12_block/5(State_iq_line_12_15_032f0), iq_bus_15_block/2(State_iq_line_12_15_d11d7)
  d_id_line_6_10_block/1(Blockout_d_id_line_6_10_40498) -> id_line_6_10/1
  vd_bus_21/1 -> d_vq_bus_21_block/2(State_vd_bus_21_a8899), d_id_line_21_22_block/3(State_vd_bus_21_3bbf1), d_id_load_21_block/3(State_vd_bus_21_5dea6), d_id_line_10_21_block/4(State_vd_bus_21_53c66)
  iq_line_5_7/1 -> d_id_line_5_7_block/2(State_iq_line_5_7_abaf2), iq_bus_5_block/2(State_iq_line_5_7_0b183), iq_bus_7_block/3(State_iq_line_5_7_dcfea), d_iq_line_5_7_block/2(State_iq_line_5_7_98783)
  vd_bus_15/1 -> d_vq_bus_15_block/2(State_vd_bus_15_568cb), d_id_load_15_block/3(State_vd_bus_15_8a842), d_id_line_15_18_block/3(State_vd_bus_15_67b4c), d_id_line_15_23_block/3(State_vd_bus_15_742a0), d_id_line_14_15_block/4(State_vd_bus_15_c6d58), d_id_line_12_15_block/4(State_vd_bus_15_2851a)
  d_id_line_27_30_block/1(Blockout_d_id_line_27_30_26949) -> id_line_27_30/1
  vq_bus_24/1 -> d_vd_bus_24_block/2(State_vq_bus_24_3465a), d_iq_line_24_25_block/3(State_vq_bus_24_1bac9), d_iq_line_22_24_block/4(State_vq_bus_24_1befd), d_iq_line_23_24_block/4(State_vq_bus_24_00c5d), d_iq_load_24_block/3(State_vq_bus_24_612f6)
  d_id_line_27_29_block/1(Blockout_d_id_line_27_29_5ee71) -> id_line_27_29/1
  iq_line_6_9/1 -> d_id_line_6_9_block/1(State_iq_line_6_9_a3af3), iq_bus_6_block/5(State_iq_line_6_9_51dc2), iq_bus_9_block/1(State_iq_line_6_9_55e22)
  vd_bus_18/1 -> d_vq_bus_18_block/2(State_vd_bus_18_3c890), d_id_load_18_block/3(State_vd_bus_18_bf8f3), d_id_line_18_19_block/3(State_vd_bus_18_26e57), d_id_line_15_18_block/4(State_vd_bus_18_e7afb)
  d_iq_load_15_block/1(Blockout_d_iq_load_15_d1c82) -> iq_load_15/1
  id_line_12_15/1 -> id_bus_12_block/5(State_id_line_12_15_e30db), d_iq_line_12_15_block/1(State_id_line_12_15_beed2), id_bus_15_block/2(State_id_line_12_15_8e417), d_id_line_12_15_block/1(State_id_line_12_15_19cb2)
  d_id_line_6_28_block/1(Blockout_d_id_line_6_28_3a173) -> id_line_6_28/1
  iq_line_10_17/1 -> d_id_line_10_17_block/2(State_iq_line_10_17_8c10e), d_iq_line_10_17_block/2(State_iq_line_10_17_a9ea7), iq_bus_10_block/4(State_iq_line_10_17_d7997), iq_bus_17_block/2(State_iq_line_10_17_8adde)
  vd_bus_24/1 -> d_vq_bus_24_block/2(State_vd_bus_24_b47e7), d_id_load_24_block/3(State_vd_bus_24_e8709), d_id_line_23_24_block/4(State_vd_bus_24_85dda), d_id_line_24_25_block/3(State_vd_bus_24_6e200), d_id_line_22_24_block/4(State_vd_bus_24_440b0)
  vd_bus_19/1 -> d_vq_bus_19_block/2(State_vd_bus_19_f463f), d_id_line_19_20_block/3(State_vd_bus_19_720ac), d_id_load_19_block/3(State_vd_bus_19_07a12), d_id_line_18_19_block/4(State_vd_bus_19_37873)
  iq_line_6_10/1 -> d_id_line_6_10_block/1(State_iq_line_6_10_1e2b8), iq_bus_6_block/6(State_iq_line_6_10_0da9e), iq_bus_10_block/2(State_iq_line_6_10_9ea7c)
  vd_bus_2/1 -> d_vq_bus_2_block/2(State_vd_bus_2_c8ab9), d_id_load_2_block/3(State_vd_bus_2_46ad8), d_id_line_2_4_block/3(State_vd_bus_2_1a8e6), d_id_line_2_5_block/3(State_vd_bus_2_fba8e), vd_bus_2_out_block/1(State_vd_bus_2_51c98), d_id_line_1_2_block/4(State_vd_bus_2_3fb4b), d_id_line_2_6_block/3(State_vd_bus_2_83f23)
  vq_bus_7/1 -> d_vd_bus_7_block/2(State_vq_bus_7_f4b0c), d_iq_load_7_block/3(State_vq_bus_7_bc847), d_iq_line_6_7_block/4(State_vq_bus_7_9b0dd), vq_bus_7_out_block/1(State_vq_bus_7_4fcda), d_iq_line_5_7_block/4(State_vq_bus_7_b0dc6)
  id_line_19_20/1 -> d_id_line_19_20_block/1(State_id_line_19_20_52ad5), d_iq_line_19_20_block/1(State_id_line_19_20_b531a), id_bus_19_block/3(State_id_line_19_20_f791c), id_bus_20_block/3(State_id_line_19_20_ee948)
  vq_bus_22/1 -> d_vd_bus_22_block/2(State_vq_bus_22_93f74), d_iq_line_21_22_block/4(State_vq_bus_22_8ed98), vq_bus_22_out_block/1(State_vq_bus_22_5efef), d_iq_line_10_22_block/4(State_vq_bus_22_cc06f), d_iq_line_22_24_block/3(State_vq_bus_22_11d1c)
  d_id_load_18_block/1(Blockout_d_id_load_18_3083b) -> id_load_18/1
  d_iq_line_10_21_block/1(Blockout_d_iq_line_10_21_9f8c0) -> iq_line_10_21/1
  d_vq_bus_21_block/1(Blockout_d_vq_bus_21_3dcf9) -> vq_bus_21/1
  d_iq_line_12_13_block/1(Blockout_d_iq_line_12_13_55f5a) -> iq_line_12_13/1
  d_vq_bus_23_block/1(Blockout_d_vq_bus_23_b171c) -> vq_bus_23/1
  d_iq_load_4_block/1(Blockout_d_iq_load_4_2d77b) -> iq_load_4/1
  d_iq_line_15_18_block/1(Blockout_d_iq_line_15_18_9343c) -> iq_line_15_18/1
  d_vd_bus_19_block/1(Blockout_d_vd_bus_19_c546e) -> vd_bus_19/1
  vq_bus_21/1 -> d_iq_load_21_block/3(State_vq_bus_21_cc767), d_iq_line_10_21_block/4(State_vq_bus_21_091f2), d_vd_bus_21_block/2(State_vq_bus_21_fbe4c), d_iq_line_21_22_block/3(State_vq_bus_21_8118e)
  d_vd_bus_10_block/1(Blockout_d_vd_bus_10_946a6) -> vd_bus_10/1
  d_vq_bus_9_block/1(Blockout_d_vq_bus_9_087a9) -> vq_bus_9/1
  d_iq_line_15_23_block/1(Blockout_d_iq_line_15_23_620f2) -> iq_line_15_23/1
  d_id_line_3_4_block/1(Blockout_d_id_line_3_4_45374) -> id_line_3_4/1
  id_line_24_25/1 -> id_bus_25_block/1(State_id_line_24_25_2e897), id_bus_24_block/4(State_id_line_24_25_6b48d), d_id_line_24_25_block/1(State_id_line_24_25_f5b6e), d_iq_line_24_25_block/1(State_id_line_24_25_c259a)
  d_id_line_12_14_block/1(Blockout_d_id_line_12_14_0b4f3) -> id_line_12_14/1
  id_line_8_28/1 -> id_bus_28_block/2(State_id_line_8_28_46f95), d_id_line_8_28_block/1(State_id_line_8_28_e35e6), d_iq_line_8_28_block/1(State_id_line_8_28_812ec), id_bus_8_block/3(State_id_line_8_28_28354)
  id_line_6_28/1 -> id_bus_6_block/7(State_id_line_6_28_5760f), id_bus_28_block/1(State_id_line_6_28_b8533), d_iq_line_6_28_block/1(State_id_line_6_28_8e443), d_id_line_6_28_block/1(State_id_line_6_28_16dd7)
  d_id_line_4_12_block/1(Blockout_d_id_line_4_12_f1df0) -> id_line_4_12/1
  vq_bus_30/1 -> d_iq_load_30_block/3(State_vq_bus_30_d32ca), d_iq_line_27_30_block/4(State_vq_bus_30_735a2), d_iq_line_29_30_block/4(State_vq_bus_30_6aab5), d_vd_bus_30_block/2(State_vq_bus_30_f82c1)
  iq_load_2/1 -> iq_bus_2_block/2(State_iq_load_2_becb6), d_iq_load_2_block/2(State_iq_load_2_ec1f4), d_id_load_2_block/2(State_iq_load_2_16be9)
  d_id_line_6_9_block/1(Blockout_d_id_line_6_9_67e91) -> id_line_6_9/1
  d_iq_load_20_block/1(Blockout_d_iq_load_20_f0a03) -> iq_load_20/1
  d_vq_bus_15_block/1(Blockout_d_vq_bus_15_2b663) -> vq_bus_15/1
  id_line_4_12/1 -> d_iq_line_4_12_block/1(State_id_line_4_12_e9a32), id_bus_4_block/5(State_id_line_4_12_0ad5f), id_bus_12_block/2(State_id_line_4_12_8182e)
  id_line_3_4/1 -> id_bus_4_block/3(State_id_line_3_4_41268), d_id_line_3_4_block/1(State_id_line_3_4_c783d), id_bus_3_block/3(State_id_line_3_4_6ece1), d_iq_line_3_4_block/1(State_id_line_3_4_c2377)
  vd_bus_13/1 -> d_vq_bus_13_block/2(State_vd_bus_13_824e9), vd_bus_13_out_block/1(State_vd_bus_13_f83b5), d_id_line_12_13_block/3(State_vd_bus_13_6c93a)
  d_iq_line_8_28_block/1(Blockout_d_iq_line_8_28_1c551) -> iq_line_8_28/1
  d_id_line_6_7_block/1(Blockout_d_id_line_6_7_5bfdb) -> id_line_6_7/1
  d_iq_load_2_block/1(Blockout_d_iq_load_2_69c38) -> iq_load_2/1
  vd_bus_14/1 -> d_vq_bus_14_block/2(State_vd_bus_14_a89db), d_id_load_14_block/3(State_vd_bus_14_f08fd), d_id_line_12_14_block/4(State_vd_bus_14_de14e), d_id_line_14_15_block/3(State_vd_bus_14_5ffe4)
  iq_line_4_6/1 -> d_id_line_4_6_block/2(State_iq_line_4_6_0a7d7), iq_bus_6_block/2(State_iq_line_4_6_7829d), d_iq_line_4_6_block/2(State_iq_line_4_6_338ba), iq_bus_4_block/4(State_iq_line_4_6_d2f2a)
  iq_load_3/1 -> iq_bus_3_block/1(State_iq_load_3_98680), d_id_load_3_block/2(State_iq_load_3_e3dcb), d_iq_load_3_block/2(State_iq_load_3_5e9df)
  vd_bus_25/1 -> d_vq_bus_25_block/2(State_vd_bus_25_5727a), d_id_line_24_25_block/4(State_vd_bus_25_6942f), d_id_line_25_27_block/3(State_vd_bus_25_03d67), d_id_line_25_26_block/3(State_vd_bus_25_d2af0)
  id_line_4_6/1 -> id_bus_4_block/4(State_id_line_4_6_c02d6), id_bus_6_block/2(State_id_line_4_6_eeef8), d_iq_line_4_6_block/1(State_id_line_4_6_aad9c), d_id_line_4_6_block/1(State_id_line_4_6_53ca8)
  iq_line_16_17/1 -> d_iq_line_16_17_block/2(State_iq_line_16_17_c5f3c), iq_bus_17_block/3(State_iq_line_16_17_d8ac8), d_id_line_16_17_block/2(State_iq_line_16_17_49d5c), iq_bus_16_block/3(State_iq_line_16_17_2d89b)
  iq_line_6_8/1 -> d_id_line_6_8_block/2(State_iq_line_6_8_15cb0), iq_bus_6_block/4(State_iq_line_6_8_410de), iq_bus_8_block/2(State_iq_line_6_8_44342), d_iq_line_6_8_block/2(State_iq_line_6_8_6bc9f)
  d_iq_line_1_3_block/1(Blockout_d_iq_line_1_3_dab4a) -> iq_line_1_3/1
  vq_bus_12/1 -> d_iq_line_4_12_block/2(State_vq_bus_12_318e0), d_iq_line_12_13_block/2(State_vq_bus_12_22143), d_vd_bus_12_block/2(State_vq_bus_12_edbb2), d_iq_line_12_14_block/3(State_vq_bus_12_dcaec), d_iq_line_12_15_block/3(State_vq_bus_12_5723c), d_iq_line_12_16_block/3(State_vq_bus_12_19670), d_iq_load_12_block/3(State_vq_bus_12_ac2a3)
  id_line_6_7/1 -> id_bus_6_block/3(State_id_line_6_7_6920a), d_iq_line_6_7_block/1(State_id_line_6_7_667e6), d_id_line_6_7_block/1(State_id_line_6_7_795b3), id_bus_7_block/4(State_id_line_6_7_ce94d)
  d_id_load_24_block/1(Blockout_d_id_load_24_7bbe2) -> id_load_24/1
  id_line_10_20/1 -> id_bus_10_block/5(State_id_line_10_20_18f02), d_id_line_10_20_block/1(State_id_line_10_20_265b4), id_bus_20_block/2(State_id_line_10_20_7e98a), d_iq_line_10_20_block/1(State_id_line_10_20_31cef)
  id_load_20/1 -> d_iq_load_20_block/1(State_id_load_20_a93db), id_bus_20_block/1(State_id_load_20_3e20a), d_id_load_20_block/1(State_id_load_20_93d05)
  d_id_line_2_6_block/1(Blockout_d_id_line_2_6_9ce60) -> id_line_2_6/1
  d_iq_load_21_block/1(Blockout_d_iq_load_21_5945b) -> iq_load_21/1
  d_id_load_8_block/1(Blockout_d_id_load_8_0e169) -> id_load_8/1
  id_line_16_17/1 -> d_id_line_16_17_block/1(State_id_line_16_17_5c8bf), id_bus_17_block/3(State_id_line_16_17_e2e89), d_iq_line_16_17_block/1(State_id_line_16_17_721a9), id_bus_16_block/3(State_id_line_16_17_d7b9d)
  id_line_12_16/1 -> id_bus_12_block/6(State_id_line_12_16_2f396), id_bus_16_block/2(State_id_line_12_16_31af9), d_iq_line_12_16_block/1(State_id_line_12_16_32f87), d_id_line_12_16_block/1(State_id_line_12_16_8024a)
  d_iq_load_19_block/1(Blockout_d_iq_load_19_8f082) -> iq_load_19/1
  d_id_load_12_block/1(Blockout_d_id_load_12_82ad0) -> id_load_12/1
  iq_load_18/1 -> d_id_load_18_block/2(State_iq_load_18_e520e), d_iq_load_18_block/2(State_iq_load_18_d8478), iq_bus_18_block/1(State_iq_load_18_b73eb)
  iq_line_4_12/1 -> iq_bus_4_block/5(State_iq_line_4_12_8cce3), iq_bus_12_block/2(State_iq_line_4_12_d3882), d_id_line_4_12_block/1(State_iq_line_4_12_530ed)
  vd_bus_22/1 -> d_vq_bus_22_block/2(State_vd_bus_22_2b8c2), d_id_line_10_22_block/4(State_vd_bus_22_ced80), d_id_line_21_22_block/4(State_vd_bus_22_0f9f9), vd_bus_22_out_block/1(State_vd_bus_22_214cf), d_id_line_22_24_block/3(State_vd_bus_22_6ca17)
  iq_line_21_22/1 -> d_iq_line_21_22_block/2(State_iq_line_21_22_2fa40), iq_bus_22_block/3(State_iq_line_21_22_a7d32), iq_bus_21_block/3(State_iq_line_21_22_832b6), d_id_line_21_22_block/2(State_iq_line_21_22_c44a2)
  iq_line_25_26/1 -> d_id_line_25_26_block/2(State_iq_line_25_26_dac95), iq_bus_26_block/2(State_iq_line_25_26_3a876), d_iq_line_25_26_block/2(State_iq_line_25_26_5031e), iq_bus_25_block/2(State_iq_line_25_26_b28ea)
  id_line_12_14/1 -> d_iq_line_12_14_block/1(State_id_line_12_14_b6e48), id_bus_12_block/4(State_id_line_12_14_017fa), id_bus_14_block/2(State_id_line_12_14_e86dc), d_id_line_12_14_block/1(State_id_line_12_14_67792)
  vq_bus_8/1 -> d_vd_bus_8_block/2(State_vq_bus_8_257eb), d_iq_line_6_8_block/4(State_vq_bus_8_0df72), d_iq_load_8_block/3(State_vq_bus_8_10b00), d_iq_line_8_28_block/4(State_vq_bus_8_f157d)
  id_load_12/1 -> id_bus_12_block/1(State_id_load_12_8eb9c), d_iq_load_12_block/1(State_id_load_12_a9fac), d_id_load_12_block/1(State_id_load_12_7246e)
  d_vq_bus_24_block/1(Blockout_d_vq_bus_24_2859e) -> vq_bus_24/1
  d_vd_bus_24_block/1(Blockout_d_vd_bus_24_09370) -> vd_bus_24/1
  iq_line_29_30/1 -> d_id_line_29_30_block/2(State_iq_line_29_30_06255), iq_bus_29_block/3(State_iq_line_29_30_aaab3), iq_bus_30_block/3(State_iq_line_29_30_a165e), d_iq_line_29_30_block/2(State_iq_line_29_30_5dcc0)
  id_load_23/1 -> d_id_load_23_block/1(State_id_load_23_139dd), id_bus_23_block/2(State_id_load_23_5361b), d_iq_load_23_block/1(State_id_load_23_359e1)
  vq_bus_19/1 -> d_vd_bus_19_block/2(State_vq_bus_19_a5c18), d_iq_load_19_block/3(State_vq_bus_19_94ea2), d_iq_line_19_20_block/3(State_vq_bus_19_a0dab), d_iq_line_18_19_block/4(State_vq_bus_19_d8da0)
  d_vd_bus_20_block/1(Blockout_d_vd_bus_20_bf639) -> vd_bus_20/1
  id_load_4/1 -> id_bus_4_block/1(State_id_load_4_57c3e), d_id_load_4_block/1(State_id_load_4_a067e), d_iq_load_4_block/1(State_id_load_4_5343f)
  d_vq_bus_17_block/1(Blockout_d_vq_bus_17_cf2d4) -> vq_bus_17/1
  vq_bus_15/1 -> d_iq_load_15_block/3(State_vq_bus_15_9de62), d_iq_line_14_15_block/4(State_vq_bus_15_80bf7), d_iq_line_15_18_block/3(State_vq_bus_15_ceac7), d_vd_bus_15_block/2(State_vq_bus_15_cc2ed), d_iq_line_12_15_block/4(State_vq_bus_15_811f3), d_iq_line_15_23_block/3(State_vq_bus_15_76336)
  id_line_27_29/1 -> id_bus_27_block/3(State_id_line_27_29_ed62c), d_iq_line_27_29_block/1(State_id_line_27_29_86314), id_bus_29_block/2(State_id_line_27_29_0ffe7), d_id_line_27_29_block/1(State_id_line_27_29_5dcac)
  vq_bus_26/1 -> d_vd_bus_26_block/2(State_vq_bus_26_91c38), d_iq_line_25_26_block/4(State_vq_bus_26_76074), d_iq_load_26_block/3(State_vq_bus_26_a53b6)
  id_line_29_30/1 -> d_id_line_29_30_block/1(State_id_line_29_30_49020), d_iq_line_29_30_block/1(State_id_line_29_30_717f3), id_bus_29_block/3(State_id_line_29_30_80eff), id_bus_30_block/3(State_id_line_29_30_b478a)
  d_vd_bus_7_block/1(Blockout_d_vd_bus_7_4e9f1) -> vd_bus_7/1
  id_line_10_17/1 -> id_bus_10_block/4(State_id_line_10_17_ef9ff), d_id_line_10_17_block/1(State_id_line_10_17_9d65e), id_bus_17_block/2(State_id_line_10_17_3b6f4), d_iq_line_10_17_block/1(State_id_line_10_17_8e75b)
  vd_bus_10/1 -> d_vq_bus_10_block/2(State_vd_bus_10_649cc), d_id_line_6_10_block/2(State_vd_bus_10_6889c), d_id_line_9_10_block/2(State_vd_bus_10_163ea), d_id_line_10_20_block/3(State_vd_bus_10_a2605), d_id_line_10_17_block/3(State_vd_bus_10_ba0ab), d_id_line_10_21_block/3(State_vd_bus_10_3ade5), d_id_line_10_22_block/3(State_vd_bus_10_b72dc), d_id_load_10_block/3(State_vd_bus_10_876fd)
  iq_line_2_4/1 -> d_id_line_2_4_block/2(State_iq_line_2_4_7f64b), iq_bus_2_block/4(State_iq_line_2_4_c1409), iq_bus_4_block/2(State_iq_line_2_4_37eb2), d_iq_line_2_4_block/2(State_iq_line_2_4_b638e)
  iq_load_21/1 -> iq_bus_21_block/1(State_iq_load_21_44508), d_iq_load_21_block/2(State_iq_load_21_200f9), d_id_load_21_block/2(State_iq_load_21_49e98)
  id_line_23_24/1 -> d_id_line_23_24_block/1(State_id_line_23_24_64227), d_iq_line_23_24_block/1(State_id_line_23_24_71134), id_bus_23_block/4(State_id_line_23_24_0bbc7), id_bus_24_block/3(State_id_line_23_24_8269a)
  vd_bus_5/1 -> d_vq_bus_5_block/2(State_vd_bus_5_28f77), d_id_line_2_5_block/4(State_vd_bus_5_3f7e8), d_id_line_5_7_block/3(State_vd_bus_5_fcd45)
  id_load_7/1 -> d_id_load_7_block/1(State_id_load_7_59ac3), d_iq_load_7_block/1(State_id_load_7_bd96d), id_bus_7_block/2(State_id_load_7_78ca4)
  iq_line_10_21/1 -> d_id_line_10_21_block/2(State_iq_line_10_21_aacb6), iq_bus_10_block/6(State_iq_line_10_21_f5701), d_iq_line_10_21_block/2(State_iq_line_10_21_3e3dc), iq_bus_21_block/2(State_iq_line_10_21_86c36)
  id_line_25_27/1 -> d_id_line_25_27_block/1(State_id_line_25_27_be6b9), d_iq_line_25_27_block/1(State_id_line_25_27_adc44), id_bus_25_block/3(State_id_line_25_27_89c78), id_bus_27_block/2(State_id_line_25_27_a3c54)
  iq_load_12/1 -> d_iq_load_12_block/2(State_iq_load_12_0eed2), d_id_load_12_block/2(State_iq_load_12_5d0f3), iq_bus_12_block/1(State_iq_load_12_bc973)
  d_iq_line_14_15_block/1(Blockout_d_iq_line_14_15_23a62) -> iq_line_14_15/1
  id_load_21/1 -> d_id_load_21_block/1(State_id_load_21_69a18), d_iq_load_21_block/1(State_id_load_21_1a39e), id_bus_21_block/1(State_id_load_21_b42be)
  vd_bus_16/1 -> d_vq_bus_16_block/2(State_vd_bus_16_b3b80), d_id_load_16_block/3(State_vd_bus_16_dbff6), d_id_line_16_17_block/3(State_vd_bus_16_c102f), d_id_line_12_16_block/4(State_vd_bus_16_dfe3f)
  d_id_line_12_16_block/1(Blockout_d_id_line_12_16_004d6) -> id_line_12_16/1
  id_line_9_10/1 -> id_bus_9_block/2(State_id_line_9_10_f038a), id_bus_10_block/3(State_id_line_9_10_7013c), d_iq_line_9_10_block/1(State_id_line_9_10_9405b)
  iq_load_20/1 -> d_iq_load_20_block/2(State_iq_load_20_f0103), iq_bus_20_block/1(State_iq_load_20_1f6b7), d_id_load_20_block/2(State_iq_load_20_02020)
  d_id_line_25_26_block/1(Blockout_d_id_line_25_26_a039c) -> id_line_25_26/1
  iq_load_23/1 -> d_iq_load_23_block/2(State_iq_load_23_3c73d), iq_bus_23_block/2(State_iq_load_23_12e45), d_id_load_23_block/2(State_iq_load_23_9ed9d)
  vd_bus_20/1 -> d_vq_bus_20_block/2(State_vd_bus_20_3ae12), d_id_load_20_block/3(State_vd_bus_20_a40d3), d_id_line_19_20_block/4(State_vd_bus_20_fc360), d_id_line_10_20_block/4(State_vd_bus_20_a0401)
  vq_bus_5/1 -> d_vd_bus_5_block/2(State_vq_bus_5_87cc9), d_iq_line_5_7_block/3(State_vq_bus_5_129b8), d_iq_line_2_5_block/4(State_vq_bus_5_87317)
  iq_load_8/1 -> d_id_load_8_block/2(State_iq_load_8_8935f), iq_bus_8_block/1(State_iq_load_8_74755), d_iq_load_8_block/2(State_iq_load_8_f08e9)
  id_line_9_11/1 -> d_iq_line_9_11_block/1(State_id_line_9_11_716ef), id_bus_9_block/3(State_id_line_9_11_17709), id_bus_11_block/1(State_id_line_9_11_37f59)
  id_line_2_5/1 -> d_id_line_2_5_block/1(State_id_line_2_5_56197), d_iq_line_2_5_block/1(State_id_line_2_5_54524), id_bus_2_block/5(State_id_line_2_5_1281e), id_bus_5_block/1(State_id_line_2_5_9c966)
  d_vd_bus_25_block/1(Blockout_d_vd_bus_25_c0f98) -> vd_bus_25/1
  vq_bus_13/1 -> d_vd_bus_13_block/2(State_vq_bus_13_d83fb), vq_bus_13_out_block/1(State_vq_bus_13_2e03a), d_iq_line_12_13_block/3(State_vq_bus_13_c3943)
  id_line_2_4/1 -> id_bus_4_block/2(State_id_line_2_4_e4641), d_id_line_2_4_block/1(State_id_line_2_4_3a3db), d_iq_line_2_4_block/1(State_id_line_2_4_7fbc5), id_bus_2_block/4(State_id_line_2_4_9c9be)
  id_load_30/1 -> d_id_load_30_block/1(State_id_load_30_f5eec), d_iq_load_30_block/1(State_id_load_30_df562), id_bus_30_block/1(State_id_load_30_9a1a0)
  d_iq_line_21_22_block/1(Blockout_d_iq_line_21_22_19dd1) -> iq_line_21_22/1
  vq_bus_11/1 -> d_iq_line_9_11_block/2(State_vq_bus_11_310c2), d_vd_bus_11_block/2(State_vq_bus_11_56182)
  id_load_16/1 -> d_id_load_16_block/1(State_id_load_16_b19cd), id_bus_16_block/1(State_id_load_16_85ef4), d_iq_load_16_block/1(State_id_load_16_bee16)
  iq_load_17/1 -> d_id_load_17_block/2(State_iq_load_17_ca59a), d_iq_load_17_block/2(State_iq_load_17_00d7f), iq_bus_17_block/1(State_iq_load_17_c996c)
  id_load_17/1 -> d_id_load_17_block/1(State_id_load_17_a4ece), d_iq_load_17_block/1(State_id_load_17_33982), id_bus_17_block/1(State_id_load_17_98f31)
  iq_load_16/1 -> d_id_load_16_block/2(State_iq_load_16_b414b), d_iq_load_16_block/2(State_iq_load_16_5f7c5), iq_bus_16_block/1(State_iq_load_16_aacc5)
  d_vd_bus_13_block/1(Blockout_d_vd_bus_13_93e1c) -> vd_bus_13/1
  iq_load_10/1 -> d_id_load_10_block/2(State_iq_load_10_46bbe), d_iq_load_10_block/2(State_iq_load_10_267fb), iq_bus_10_block/1(State_iq_load_10_2c7ec)
  vq_bus_9/1 -> d_vd_bus_9_block/2(State_vq_bus_9_a0ae4), d_iq_line_6_9_block/3(State_vq_bus_9_a086b), d_iq_line_9_10_block/3(State_vq_bus_9_3ff0d), d_iq_line_9_11_block/3(State_vq_bus_9_0d25d)
  d_id_load_19_block/1(Blockout_d_id_load_19_c7816) -> id_load_19/1
  vd_bus_8/1 -> d_vq_bus_8_block/2(State_vd_bus_8_8cd22), d_id_load_8_block/3(State_vd_bus_8_e6dd7), d_id_line_8_28_block/4(State_vd_bus_8_26ad6), d_id_line_6_8_block/4(State_vd_bus_8_3fe16)
  d_vd_bus_2_block/1(Blockout_d_vd_bus_2_2c7da) -> vd_bus_2/1
  vq_bus_3/1 -> d_vd_bus_3_block/2(State_vq_bus_3_0fb23), d_iq_load_3_block/3(State_vq_bus_3_cb59e), d_iq_line_1_3_block/4(State_vq_bus_3_23559), d_iq_line_3_4_block/3(State_vq_bus_3_53dc7)
  d_id_load_26_block/1(Blockout_d_id_load_26_29eef) -> id_load_26/1
  d_vd_bus_26_block/1(Blockout_d_vd_bus_26_d635e) -> vd_bus_26/1
  d_id_line_24_25_block/1(Blockout_d_id_line_24_25_64f9d) -> id_line_24_25/1
  d_vd_bus_22_block/1(Blockout_d_vd_bus_22_f19b2) -> vd_bus_22/1
  d_id_load_30_block/1(Blockout_d_id_load_30_6a7a7) -> id_load_30/1
  d_iq_line_12_16_block/1(Blockout_d_iq_line_12_16_07cfb) -> iq_line_12_16/1
  d_iq_line_16_17_block/1(Blockout_d_iq_line_16_17_36e2b) -> iq_line_16_17/1
  iq_bus_9_block/1(Blockout_iq_bus_9_1e267) -> d_vq_bus_9_block/1(Alge_iq_bus_9_8054c)
  d_id_line_2_5_block/1(Blockout_d_id_line_2_5_534b8) -> id_line_2_5/1
  d_iq_line_6_10_block/1(Blockout_d_iq_line_6_10_02488) -> iq_line_6_10/1
  d_iq_load_17_block/1(Blockout_d_iq_load_17_3c8b9) -> iq_load_17/1
  d_id_line_14_15_block/1(Blockout_d_id_line_14_15_f4e19) -> id_line_14_15/1
  d_vd_bus_14_block/1(Blockout_d_vd_bus_14_5026c) -> vd_bus_14/1
  d_id_line_15_18_block/1(Blockout_d_id_line_15_18_32fdd) -> id_line_15_18/1
  d_iq_line_3_4_block/1(Blockout_d_iq_line_3_4_9b5ec) -> iq_line_3_4/1
  d_id_load_23_block/1(Blockout_d_id_load_23_0d04d) -> id_load_23/1
  d_id_line_19_20_block/1(Blockout_d_id_line_19_20_50907) -> id_line_19_20/1
  d_id_line_15_23_block/1(Blockout_d_id_line_15_23_c2a70) -> id_line_15_23/1
  d_id_load_7_block/1(Blockout_d_id_load_7_06d7e) -> id_load_7/1
  d_id_load_21_block/1(Blockout_d_id_load_21_f09db) -> id_load_21/1
  d_id_line_1_2_block/1(Blockout_d_id_line_1_2_c33ff) -> id_line_1_2/1
  d_id_line_1_3_block/1(Blockout_d_id_line_1_3_0fd49) -> id_line_1_3/1
  d_iq_line_10_22_block/1(Blockout_d_iq_line_10_22_034e5) -> iq_line_10_22/1
  d_id_load_20_block/1(Blockout_d_id_load_20_0f852) -> id_load_20/1
  d_id_line_21_22_block/1(Blockout_d_id_line_21_22_f50b1) -> id_line_21_22/1
  d_vd_bus_5_block/1(Blockout_d_vd_bus_5_739c0) -> vd_bus_5/1
  d_iq_line_10_20_block/1(Blockout_d_iq_line_10_20_deb13) -> iq_line_10_20/1
  d_id_line_5_7_block/1(Blockout_d_id_line_5_7_7d91d) -> id_line_5_7/1
  d_id_line_25_27_block/1(Blockout_d_id_line_25_27_d028e) -> id_line_25_27/1
  d_id_line_29_30_block/1(Blockout_d_id_line_29_30_18eb7) -> id_line_29_30/1
  d_id_line_2_4_block/1(Blockout_d_id_line_2_4_f10ed) -> id_line_2_4/1
  d_id_line_4_6_block/1(Blockout_d_id_line_4_6_c5916) -> id_line_4_6/1
  d_id_load_10_block/1(Blockout_d_id_load_10_a9a8b) -> id_load_10/1
  d_id_line_8_28_block/1(Blockout_d_id_line_8_28_c2b8a) -> id_line_8_28/1
  d_id_load_29_block/1(Blockout_d_id_load_29_ee930) -> id_load_29/1
  d_id_load_14_block/1(Blockout_d_id_load_14_6d751) -> id_load_14/1
  d_id_load_15_block/1(Blockout_d_id_load_15_10a9e) -> id_load_15/1
  d_id_load_17_block/1(Blockout_d_id_load_17_000e5) -> id_load_17/1
  d_iq_line_1_2_block/1(Blockout_d_iq_line_1_2_85e11) -> iq_line_1_2/1
  d_iq_line_6_9_block/1(Blockout_d_iq_line_6_9_e28b1) -> iq_line_6_9/1
  d_vd_bus_29_block/1(Blockout_d_vd_bus_29_ae863) -> vd_bus_29/1
  d_id_load_3_block/1(Blockout_d_id_load_3_d01d9) -> id_load_3/1
  d_iq_line_10_17_block/1(Blockout_d_iq_line_10_17_34a6b) -> iq_line_10_17/1
  d_iq_line_18_19_block/1(Blockout_d_iq_line_18_19_0dac2) -> iq_line_18_19/1
  d_iq_line_2_4_block/1(Blockout_d_iq_line_2_4_be6c7) -> iq_line_2_4/1
  d_iq_line_27_30_block/1(Blockout_d_iq_line_27_30_4beb9) -> iq_line_27_30/1
  d_iq_line_24_25_block/1(Blockout_d_iq_line_24_25_5a1b9) -> iq_line_24_25/1
  d_iq_line_27_29_block/1(Blockout_d_iq_line_27_29_c732b) -> iq_line_27_29/1
  d_iq_load_29_block/1(Blockout_d_iq_load_29_f93a9) -> iq_load_29/1
  d_iq_line_28_27_block/1(Blockout_d_iq_line_28_27_81b11) -> iq_line_28_27/1
  d_iq_line_29_30_block/1(Blockout_d_iq_line_29_30_05166) -> iq_line_29_30/1
  d_iq_line_2_5_block/1(Blockout_d_iq_line_2_5_eff7c) -> iq_line_2_5/1
  d_iq_line_4_6_block/1(Blockout_d_iq_line_4_6_3cc9a) -> iq_line_4_6/1
  d_iq_line_5_7_block/1(Blockout_d_iq_line_5_7_5e840) -> iq_line_5_7/1
  d_iq_line_6_7_block/1(Blockout_d_iq_line_6_7_6dbe9) -> iq_line_6_7/1
  d_iq_line_9_10_block/1(Blockout_d_iq_line_9_10_d1a46) -> iq_line_9_10/1
  d_vq_bus_19_block/1(Blockout_d_vq_bus_19_831b3) -> vq_bus_19/1
  d_iq_load_14_block/1(Blockout_d_iq_load_14_e1c59) -> iq_load_14/1
  d_vq_bus_11_block/1(Blockout_d_vq_bus_11_520df) -> vq_bus_11/1
  d_iq_load_23_block/1(Blockout_d_iq_load_23_36f94) -> iq_load_23/1
  d_iq_load_3_block/1(Blockout_d_iq_load_3_3c3bc) -> iq_load_3/1
  d_vd_bus_11_block/1(Blockout_d_vd_bus_11_c002c) -> vd_bus_11/1
  d_vd_bus_15_block/1(Blockout_d_vd_bus_15_eaf4b) -> vd_bus_15/1
  d_vd_bus_17_block/1(Blockout_d_vd_bus_17_9b1fc) -> vd_bus_17/1
  d_vd_bus_1_block/1(Blockout_d_vd_bus_1_200d9) -> vd_bus_1/1
  d_vd_bus_23_block/1(Blockout_d_vd_bus_23_d2881) -> vd_bus_23/1
  d_vd_bus_4_block/1(Blockout_d_vd_bus_4_76e25) -> vd_bus_4/1
  d_vd_bus_27_block/1(Blockout_d_vd_bus_27_83d7e) -> vd_bus_27/1
  d_vd_bus_3_block/1(Blockout_d_vd_bus_3_b5880) -> vd_bus_3/1
  d_vq_bus_16_block/1(Blockout_d_vq_bus_16_2931f) -> vq_bus_16/1
  d_vq_bus_18_block/1(Blockout_d_vq_bus_18_0ee5d) -> vq_bus_18/1
  d_vq_bus_20_block/1(Blockout_d_vq_bus_20_225c5) -> vq_bus_20/1
  d_vq_bus_25_block/1(Blockout_d_vq_bus_25_e403d) -> vq_bus_25/1
  d_vq_bus_27_block/1(Blockout_d_vq_bus_27_9b6db) -> vq_bus_27/1
  d_vq_bus_29_block/1(Blockout_d_vq_bus_29_9ca95) -> vq_bus_29/1
  d_vq_bus_2_block/1(Blockout_d_vq_bus_2_d5528) -> vq_bus_2/1
  d_vq_bus_30_block/1(Blockout_d_vq_bus_30_e3d22) -> vq_bus_30/1
  d_vq_bus_4_block/1(Blockout_d_vq_bus_4_757f0) -> vq_bus_4/1
  d_vq_bus_8_block/1(Blockout_d_vq_bus_8_7917f) -> vq_bus_8/1
